simulink model "Noa_Nofusion"  (R2020b)
settings: Solver=FixedStepDiscrete  StartTime=0.0  StopTime=Inf  FixedStep=0.01  RelTol=1e-3
PostLoadFcn:
  | if any(exist('dsrtsu_mdlpostloadfcn', 'file') ~= 0), dsrtsu_mdlpostloadfcn('Execute', bdroot); end
InitFcn:
  | , if any(exist('rtifpga_mdlclblib', 'file') ~= 0), rtifpga_mdlclblib('Init', bdroot); end,
  | , if any(exist('dsmpb_private', 'file') ~= 0), dsmpb_private('dsmpb_mdlclblib', 'Init', bdroot); end,
undefined symbols (not defined in the file or in its folder): ACC_TimeGap_DecSetSwt, ACC_TimeGap_IncSetSwt, AccelPedalPosn, AccelPedalPosnVldty, AccelPedlPosnDiagc, AccPedalOverride, ACU_ShiftInProgress, ADAS_Posn_CurLane, AESSwtReq, ALC_SwtReq, BrkPedalSts, CC_ACC_CANCEL_OFFSwt, CC_ACC_CRUISE_OFFSwt, CC_ACC_DecSetSpd_SetSwt, CC_ACC_IncSetSpd_ResuSwt, CC_ACCSwtErr, CharSpd_ms, CSA_NODE, CURRENT_GEAR, CurrentGearValid, DiscIntNeverNeededParam, DrvDoorSts, DrvSBR, DrvTrqReqOvld, ECMACCInterface, ECMRespACC, ELKSwtReq, EngLimpHomeSts, EngSpd, EngState, EngState_PHEV, EngTrqMaxActSpd, EngTrqMinAct, EPS_DrvInpTrqVal_HighReslolution, EPS_FailSts, EPS_LKATorqOvrlDlvd, EPS_LKATorqOvrlDlvdVld, EPS_LKATrqOvlDlvdSts, EPS_SteerMod, EPS_TrqSnsrSts, EQ4_APPINFO, EQ4_LA_ELEM, EQ4_LA_HDR, EQ4_LAP_ELEM, EQ4_LAP_HDR, EQ4_LH_ELEM, EQ4_LH_HDR, EQ4_LRE_ELEM, EQ4_LRE_HDR, ESS_PedSwtReq, ESS_VehSwtReq, FFogLmpSts_F_Pbox, FLWheelDriveDirection, FLWheelSpd, FrntWiprSwtSts, FrntWshrSwtSts, FRWheelDriveDirection, FRWheelSpd, HazardLmpSwtSts, HCU_AccelPedalPosn_Diag ... (+151)
libraries: simulink x144, dsmpblib x33, canfdmsglib x10
(part 1 of 20)
PreSaveFcn:
  | , if any(exist('dsmpb_private', 'file') ~= 0), dsmpb_private('dsmpb_mdlclblib', 'PreSave', bdroot); end,
CloseFcn:
  | , if any(exist('dsmpb_private', 'file') ~= 0), dsmpb_private('dsmpb_mdlclblib', 'Close', bdroot); end,
settings Model: DataDictionary=HWA_DDs.sldd  RTICANMMDATA=struct('GeneralSetupData',struct('modelroot','F:\05_dspace_Work_Files\11_HWA_Project\Git_ADAS_Store\projcct\adas_project','generalsettings',struct('filesettings',struct('destfolder',struct('Name','RTICANMM_FILES','Check',1),'buildfolder',struct('Name','.','Check',1),'AbsDestfolder',struct('Name','F:\05_dspace_Work_Files\11_HWA_Project\Git_ADAS_Store\projcct\adas_project\RTICANMM_FILES'),'AbsBuildfolder',struct('Name','F:\05_dspace_Work_Files\11_HWA_Project\Git_ADAS_Store\projcct\adas_project'))),'options',struct('addpaths',1,'rmpaths',1,'addtrcexclusion',false,'cannavigator',struct('checkmonitoring',0),'show_usrtrc',0,'use_usrtrc',0),'advanced',struct('options',ones(1,100)),'MPSetup',{{}},'RTI',struct('Type','DSRT','Ver','4.4','Date','02-Nov-2020'),'modelname','Noa_Nofusion','block','Noa_Nofusion'))  DSRTSU_INTERNAL_RTIFPGA=170  DSMPB_ID_DATA={'108889',struct('BlockId','81ba8c02-39a0-4bf8-971e-fc8bc9e1d8b0','SignalIds',{{'e6dae809-112a-4cbc-98f9-354c12187ac1','31d2deb7-ef93-4695-993d-314bc5bcc843','62343d78-d15a-4a45-8693-ba2849e89479','c13156af-d15b-4771-8a29-b8e73d565fa8','cbe04a47-fa20-4770-9bbd-4a07b568eb2e','59e00f7c-c03d-4b80-a5ec-a7b536bc6272','3f246c43-0baf-4388-bea8-c24249e8d124','05e7c6b4-9822-4e1b-91fa-c2d47c80a9dc','3c91b297-0034-4136-9460-a9a71fb1b160','b0eda23f-b1b7-44f7-9430-f2199b0de4f6','d9349f60-73fd-4e07-90cc-b8a5cfade7d1','f893d12f-c8e5-49d5-ab09-89fc2cdbf4b7','b489956b-9fe5-4db2-8485-d07366cb4569','0fd99c70-4fef-4ffb-8340-8501f6b1f5e4','53dd6ff7-6c1a-46a1-9139-61ea4f9d24e0','93fe1b5e-8abc-49f2-ae51-04c114465812','9444d888-9a75-4226-ace5-9b052183c8c8','ce7a08f7-cc95-444b-9a6f-cd5054dc142c','683a3bb5-05b9-4d71-b570-d34d769ae407','6e290ea9-9348-4509-bbba-48e715a1ad64','385761be-a1f9-4d98-b926-1efaecbe94cf','77479779-8c39-4f5c-be4f-4246b8ca51ff','094c4e00-d8db-4561-82fa-1990a2a46c70','8fedcf21-59e1-4a11-b24b-5edc3eea11e5','de2ede37-26b1-45c0-988c-7281b852313f','ed4cfff0-74cb-4a5b-9058-099c9444dc97','d8a92eb8-77b2-47c6-a14b-19e5a6c1880a','bb80831f-ec06-46fe-9a60-525cce3db11c','089a9e8f-4e14-4d97-a75c-e18256b8f73e','116e4020-4c03-4eaa-a133-5105e1ad6c2c','5d390f2c-fbfa-4acc-8e45-8a78ede6d630','e0ea540d-a3ce-47e8-9630-4c2a7c2611e9','1338e80f-eb11-478f-b148-febac8b5f561','40cb9f5e-abe1-4c5a-91b1-6a21a87629f0','f68eb2ae-9d65-4ce4-8ae6-7911307f53aa','90ccc115-d294-448b-be51-2f0d4ed4df75','d061fb9a-9168-48d0-bfc4-e7fc980285e5','66fbeac1-5405-448b-aaf2-b3b4c802c6b3','18d32c7d-1106-4865-b268-b9839028e3ed','68ea3199-eee5-4804-a61b-b9492c15cc17','251bf7c6-0b5c-4442-bed5-124eaca4f0a3','5c44ff7b-7cde-47e3-997c-d7e4d571a688','a318a3ac-fb11-4e42-abce-b283a20da434','8ac8bf9e-cc00-4453-b1d3-1d8cb9e4d5f3','e889ec5a-b6bf-4115-bfb4-789ddcbb1b39','843277e1-c8e1-4956-bb5f-69810b3fca13','8015402b-cae2-47f5-b799-3258863f20da','967f47db-98cb-4b9d-8737-8d02120e8039','408e6371-4b24-4e9e-8575-3f5fd9116599','0add38a7-641b-41d0-9036-40ff81d44c7c','42c9e777-d5c1-4821-b220-ee42a71da039','1eccc895-bd9f-4c89-9169-915b3accee5d','c32a22ec-25cc-4381-9457-3401f3ef52f2','dadafd58-4047-4fbe-8c61-d0d4f2e948e4','33df5bd2-20b0-4ead-bd24-c6cd609c4787','a6ef951d-803f-431b-afeb-b8db87ab93f4','3d89e518-12b9-4d0d-90f2-936f61a4e4f2','f4fba2eb-28a8-4b3f-a3d3-e6a85bead6df','1bbb28d7-2fef-43d6-b55d-c5356e90e304','46c1d4d9-bf71-419d-bdfe-9c3255f570d2'}}),'112056',struct('BlockId','6913c789-035b-4c0b-bbc8-df30b7210019','SignalIds',{{'6e67b619-d0e1-4489-8e12-cbb641b6930f'}}),'112939',struct('BlockId','bd32a928-034f-4d93-abe8-55cc1037974b','SignalIds',{{'ed378323-8937-4e58-90a7-af861033d965'}}),'112945',struct('BlockId','c5ed9ac9-a557-4e9e-b1b2-178e2ab00d3a','SignalIds',{{'9bf7ab65-611a-4ce6-8553-94d5ebac5e02','125861c6-7b90-4e8d-a590-5d6d82b8a9a7','4aee84b7-a55c-4fa5-a4b0-5c93a3e16834','bd31e0e7-f9ed-4a3b-9100-c48940e83979','f56bb652-89fc-4dda-9d9a-1212207cf3a7','0e2341be-0c6f-46b5-93e3-ba9acd4843ed','91d7f4b2-8cda-4163-9f74-f5dfcbc91f25','b0e338de-3225-4d50-a22b-4e417233ad31'}}),'113655',struct('BlockId','cf6f5b87-7341-43e1-a3e2-6f8acef19396','SignalIds',{{'fb5a5d6d-2525-41ca-b3f6-99d6346c30ea','ae8d4c22-9733-4a6c-b1e0-ca44fb9aed0b','e1e4207b-e7d4-4434-90ef-6db7c466bdcc','10f1d399-af2e-4f78-9956-e1f0397ac4ad','4b9c207b-4222-4e4c-a939-fa1aa9ebbaa6','60cb540e-4d8e-4be8-b719-3a1a079b86f3','7a6de52f-e056-439d-aa5f-cbeab7f01795','aef0510b-cc97-44dd-85d0-c0d01358d9a8','81128469-f06a-4068-854b-26757f57e96b','bef5065e-4128-4abb-aea9-c2d2196590d7','71c1176d-d27b-4ef0-b058-205366da91eb','a3f3e7d6-0f7e-4984-a2f1-0321a3d087c0','b8f4f6e5-954b-4f58-98d6-66ac20499b5e','1b7b5941-9f2a-477b-be19-44adcd6fa043','0aca1d39-c4d5-45fe-b4c4-9737676b57c1','e506b680-642d-4f46-a400-b635b37ea192','c25a201b-c2c5-487a-9976-20a56153ab24','f54c3c26-ca72-4882-a2bb-5b3ec148117f','92e7bc4b-0bc3-4bce-8cc2-cf8f985c98ee','153941b6-b33b-4fe1-a541-d5210f1cf000','89f9b2c0-1175-4586-8022-f8668d534196','2e6f805d-9e7b-45c9-86c4-bb39c1b2e16f','812564df-09e9-4888-95e9-ea67c66976c9','ad32a513-90be-4e6f-8d45-3c98afd525bb','6bf7cf6c-3db5-431a-aa46-6683249e747d','d0d3bceb-ccfe-496f-bad6-d5b74e8fe321','28d4a00c-23a7-4c5a-a473-39ff0814a4a6','cb76da0e-2e0f-46bd-b5e5-f0a979fc9b56','dbfa4afa-9e88-4515-b868-620e1ca4efcb','9069fd4c-b476-4ee9-ab6f-15984b4dcbc6','7aa0c299-49d1-4bff-bafb-8f8a0898bcb9','41a89758-675e-48c8-b1f5-09ddc1e1d587','88f85f3d-145f-48e8-bc36-fa5a99545391','17419447-9e4a-42e5-a167-9f836768a643','7afdf13a-9d25-4c4d-8007-226f9de8ca9e','59952105-0e5e-4efa-ab7b-4572f1fda11f','c96169fe-d7f6-4165-b1ad-2f304687a6e6','24738832-79b4-4001-8229-260d8feb4113','86b2b6a5-44b0-46be-a990-c83a6a69628a','440d9c51-e2b3-4545-96e6-96bbb804c01f','2c6095e2-8169-4ae4-a16f-79f403295a42','cadb492c-0473-4401-be06-10367d0aa2ef','4e68f589-c74a-49e1-ac92-78db45f8ef8c','77831aa9-1b69-45e9-bbee-3b14b9e34578','f5305063-53ac-4dc8-9054-75ad211f45d6','5ac2eb62-480b-424b-b3fc-c0796833d037','baf4b3ea-4bfa-41be-a1b1-216d8e77a452','5a3c4cf6-1180-4e87-8a7b-237d3d652526','d1686968-86ee-456f-911e-0d6de43751eb','166edc4a-1ea0-4644-9293-bfcbe463d6ad','20e7c49e-9ca2-46af-acd9-1232cce0faa2','2fe2470b-9364-4832-b69f-2e5d9d6c017d','2429babe-f40e-4f87-8c9e-2b0729d1c86f','36be9472-502d-461e-af19-fcd14b7c07d0','4c6963a3-b37c-41a1-b24e-c4c74fe8b70e','017cf1c2-cd81-4f79-8072-322d3a102b1a','00c4aaec-f88f-44fe-9513-f362b17663da','92dd9569-6fd6-4cf3-881a-10befd4b7a04','110c0564-d01b-42f2-8faf-9704e9fd9cd7','1a8a2e8a-c290-465a-a25a-8437cce6393a','98a367f9-c024-42c5-8458-b1267635b2fe','9c1fd1a9-d357-436b-b199-147a0771b5d9','70dc3328-065a-48ed-abfc-2992969b08cb','0fb59dfc-84c6-493b-a389-3fb28a6d9fe1','0f4a0327-4eba-4d80-9017-dba17db1341e','8cc82210-4aa3-44d9-869c-a0209d9ebe66','dc67f717-48c7-4ce0-9dcf-e91aac01697b','01d17e0b-0a8d-4114-bd9c-6b82437e2631','c90d70b0-ad54-4755-b5d8-75e9be712e4e','cf4155ec-ad34-476e-ac0d-8e69f7d22b3e','b127da2b-81a2-492a-9a1d-7dde354402b7','7f843f67-d354-4c08-b6af-2ff3e43672c5','f4418185-a712-42cf-8d77-411d214ab81d','59e3a284-6d51-47b6-969e-f6b4d8174f3d','b8e8aa68-fd96-4202-895b-fd402c9a1341','5fa25c56-4452-41bc-acca-9957ac1b4103','13cf6133-db9d-489e-8b0d-61e9b3419fae','71c8cfac-5807-43ef-a652-22095fc79882','15c70bed-afca-4d00-ae5e-dd51784e9f61','aee1c38c-6fb3-4ddb-a252-226dfbfb6422','7168a0ae-fcdc-4521-b98d-6a441943bf9b','5dd8b7ac-f364-465a-a93c-c9343301ac44','df0fde16-8f04-458b-a7c8-834de1c017b8','3a947018-17ad-4272-ae69-eecc79aa5a06','cd4f05ea-2a10-442f-b08c-e22eaeb8013d','cfd99e2b-6a05-4d37-bc51-f59eebfa85f5','aa629df3-c01f-49de-b905-c90313b21dc2','22d01045-bbb1-4d02-b693-732a6fc069ae','c48275b5-fc3c-4e5d-a241-e78a85a3ad8c','c56eb02a-4f36-41d4-b430-a4b28301ef5d','bae3b75d-9e5b-4327-b68f-a846466c9a9f','400fe431-6ea0-4473-a63f-9ef8d119722a','02db0c0b-dc19-45c7-8838-2e3a10b74905','48aa7831-7c07-4a00-8123-89d3d6d7594a','bf73eca7-8306-4a9e-b009-9c4be8fbd534','d538498e-adef-4247-9bcc-456a97e2113b','d0492371-75a9-4227-9ab1-7e8aa07d4fa7','115c5825-4fd6-4e7c-bdc5-7fe3051c0051','ed0f82ce-ae1d-401f-a42a-e322d0793cbf','aa1610ed-12f6-4ed1-aae0-3315b1eb3f84','63583f44-8eb9-41d6-b0a7-68eac98b41b5','c96f8dbb-26c7-435d-9572-792809250d8d','f1980f8c-e4af-4d1b-8b98-9d32743e8941','a4369ee8-1173-4fa4-9ee3-615cb3251022','90c0388b-7c95-4d96-b447-7c88a50c7164','173dbe10-46e5-4294-a3ec-3e0e30e5a6b6','529d5fb7-0bae-43e1-b06c-704af90a34cb','3c503139-d85c-4ae5-a8e2-dee622a6f9fc','d16ad6ae-6cac-4f83-aed0-121895af10f1','f6e64590-8c21-4a07-bb10-99a1519377b0','ac732596-2512-40c1-b579-190acdd8e089','9816bf99-2d8e-44e7-85d1-d4b65f13525d','fbf136a3-9574-45df-80c7-da1f97b5e35e','a12166d6-84f5-4f22-8379-ecc27ba6ae9c','55221980-234a-42fd-aec1-f26d2630223d','f2f07aaa-464d-4e08-bbee-41e72004ebfb','03cc4663-40e3-4a19-a510-51aa2d1d5c81','c6d48439-bfbd-48e6-ad19-a014aaf6d7a4','26888429-99ef-40be-9301-8bbe11f917c8','965f7110-f95b-498e-815e-73cc2d6d6525','f2d198cc-4bd4-47b3-8c41-c7e19266237c','0eb6f2be-800e-485c-a213-fc91674a796e','14566c8d-2b3b-475d-9ec4-34982939edda','b1531aa6-8f0c-4ac4-9759-53039e63bf9b','f03e1eca-afbf-4e5a-a201-deca4b0487b3','1fd091fe-0624-4b60-9f3a-d13954dedfee','f86c37b6-0788-4db1-b32a-02556a39e0dc','eb622d94-f642-41f2-ae16-5748dc9eca3c','f552e8bf-3199-4d81-be32-9694985eedf8','89df7002-4106-4bc4-8041-9f53e3d16869','212e5966-27e2-4926-a8e7-97e15aa44966','d800a550-6f5f-4611-be9b-77cb4f1d501d','7c97f8e2-f557-439c-b46e-1b618bee852c','ba8c36d0-0984-4461-a832-bfa5f921dfb5','06934513-6eda-43e5-9ba7-043c69abb13f','00daf677-ba6e-4866-aeb4-cdb14cc8e0b9','078b0d6c-c412-49d2-950e-bbe655339b57','239e3cc7-790d-4097-9a56-e63ab309039e','66b7e7ad-a98f-4fbc-9e25-0dac0827d61c','315dca2a-b23e-4eb3-9e0b-52140b0168ea','b6365e66-fb75-4629-937b-80d218075377','9b529c23-3902-492a-874b-28d45a35fcaf','9353632c-29da-42c0-b854-eedca60acfed','b766848c-b98e-4e0d-8440-f607563ba8f6','794edea3-10a5-4aec-a36f-e1459d729f91','43984543-8420-4c46-a3e8-2d784edb7c6b','ab504fde-7461-4895-9a45-667a2b575a53','6bc6eec9-68dd-49c5-8569-ec45206b9a33','bc6a11cb-2543-455a-8027-a475be328250','8cbc4c4c-4bcd-4e64-a3f2-8b1ead7218ef','5007b9e2-cba9-4a18-8f0c-5063bf4128a5','2aad26d1-b92c-4482-b26b-b7acf4fc1308','95f5773a-c7bb-44a0-a919-27ddf233286b','9e8d56c1-5230-4c79-9a8a-dc1b7934edc1','60a91cf0-0afd-46ad-ae58-fb1a2eb831b9','4c89a1ec-5f31-4d14-a287-1ccabed8a64f','c7b205df-5cce-4a4e-ba20-1c4bdae77031','c5981b5b-3b20-4a4d-9505-1eac419a8f7e','6f213db0-4ffb-4883-a14a-5b45ff58725c','2a8d3af2-5809-4f7d-89e2-80bde3f8ad32','ed1c9b94-0fa4-4bb0-a2fe-4bb286367636','4a796490-b3d9-4bba-a58b-74691b8b9c45','3e10f08b-c794-4285-b936-32a0f1309fd3','83fda9a6-ac79-4c7f-9344-c587036b236b','1cc4289d-4d7a-4fe6-bdb5-f78a307c0c9f','b5275e4f-1cc7-4a3d-b6fe-0b4189fb04a4','2e56446c-c333-4276-95a7-367f5c85c84f','e3b40b68-b9f0-4ec0-9836-b744d2e81a25','6dc5b3ee-34ab-4f3b-8a90-542aca188307','19fe3b5f-6175-40e8-91df-5be10690c48a','bcc012ad-6a8f-4b49-9a64-37954720d3ac','140a9a36-67c9-4b06-8b1a-2c2bdb5987e8','a03085eb-5191-4509-9a9c-9f34d876ca3b','5f4143a3-b004-4871-8e65-77221395668b','86ea935d-0a1e-423b-bc47-02ae6b6a212c','6baf03a1-b91d-40eb-bce4-0ea061e1b9eb','54d848f2-396f-4317-bd62-e251125d29aa','19f4b235-e4a4-4b72-b459-b188be453e53','5343c8e3-0bf6-4584-9728-1ffdf78a1c68','60ad3be9-877a-4b12-844f-f4d858a22658','adcf0bd6-8038-4d49-afc5-721d0c718c63','fe594a46-7e27-445e-829e-e368b2766e07','34b661d0-722a-48f9-9697-2658f24a22b0','06588917-d49b-4cf1-8374-3b911c00cde5','5c34855b-78d4-4797-82d5-4cf4fb5597c2','08cc61cd-138e-4046-a793-e08ba6951309','a0299fef-0823-42f0-8309-d7777acbc38a','e0a15817-9b40-4e70-969e-86236bb9f230','9c56c4dc-6508-438a-b106-2303bc6695c3','dba36f32-39ac-41b6-9312-d45812cf79de','2d770f77-49bd-4944-b036-dceda0114cb0','d649385e-2647-4aa9-9434-450787e207f3','aea55e49-0b3c-4de1-bd15-8d3a264bed41','bce569b1-2dcf-474d-b5f0-eaaba8306cd3','188b79e3-5a90-4177-a30c-289bee269920','bedbb28f-052e-4eaa-a863-033c9bf7d025','5061b3f3-9e4c-411f-a66c-77787e28b206','16d831e7-1cc8-4971-b147-7b6dd9f1e240','602d497b-3413-4be2-a3ae-0627235695d9','b5052d5b-ffb5-4989-a31d-1768a8ce989f','a859376c-290e-4574-ac12-3aa5aeaca50e','64528274-e7f3-4fe7-823e-a549b5173330','e7e53007-1b26-4631-b4f0-90657a77a9ca','5bf9ee21-94d6-40cd-a889-88d08a7a87e5','9a38031f-a864-42ea-8e2f-b35739f9c0da','e7cb1bc1-e249-4a65-b9af-f693524c4367','b5764df3-fce9-4fba-babb-0c3ebb3c0ff9','67fa94ff-08fd-4a02-8dfe-1b7ce6c0e586','1d55abc3-0a99-4ac4-9732-7251d21b101b','03ca9ed0-8b4f-4eec-9e40-39a068e3fea1','692ec90c-8e9b-4031-84bf-366e08f2da13','be841484-f40e-46bc-9894-07f688db3a45','47930925-babf-4f1f-abbd-2ff62ce38353','64ba39f6-08d5-4ebc-9f32-4871ca2ba973','f69b6ed1-4854-4198-b013-d82baaa470cb','23d63867-9c16-4ada-a94a-83a465157190','b20f84ea-82e2-4769-80ec-cf58304b0510','8ecc5c53-55c9-498b-b349-bf6ab70d66eb','e6a2b593-080c-4bcf-8d98-d1bebd736166','aca64f4d-8f9c-4329-bd12-0bf755dcf6b2','541ff6fc-3cb8-431a-ab40-7a0072923e88','6a467d04-2bf3-4197-80f5-111fd640a6b8','388c2691-3673-42af-a5bc-3881b21e8e4a','58794cec-c59f-448f-a084-9559b6fdbc3c','53969dc3-67ba-4150-8c28-2139dcd36ec4','b047deac-9e80-4433-acac-cbf23acc33d7','893ee9b8-2597-4f15-875e-3c3b30945b0e','e6ddfd0c-2f8c-4b29-8e36-05c9546fe401','d98547d0-f670-4ea4-b98a-9385d86c2203','3b07b467-bd0e-4454-bb9a-90d280d34652','bf33618c-d18a-466d-a60d-60ac0c9409f1','775e1b57-a066-47f3-8cff-496f01feada8','eaf30c55-fe96-4594-8469-a63fc7e3cc74','c79fb195-18a4-44a3-ad68-cec237ffcfbb','ed0574a8-f84b-402a-8e0a-efcd9c69260f','3be3ed0e-9f1b-411a-a012-2e23b6931244','9d2f5e3a-9477-454b-bc3a-5f933716ee7e','8eb59546-6e82-4fa8-bbb0-53768d49ea0f','e6d25c3d-5af7-4b2e-a6ea-e57a6a9082fc','ccd97ab0-e4ee-4603-94a4-f590f332a0a0','36ec9cb7-c0de-4262-bfdc-48de79f1ee61','efb2231a-227c-4972-8174-d25c5af76b54','b8657e90-21cb-4618-9e22-eaf8199bac0a','ab860674-1233-4d97-baed-976b22bdb396','86e17527-957b-4763-8fcf-1efdfe4bf5e3','8976db8a-c2a3-4c2d-94d2-ed11fa88995e','fe62eeb1-fc5f-480b-8fcd-625981641e99','98479ede-546b-4ce3-9131-f97f4f44b420','455c1b0e-8996-46e3-8765-b54392466814','eecd774d-9fd7-4e12-a69f-9158539ea43f','64e999d6-79ea-4c70-9691-0f70a2e71a3c','4f106621-85e0-43b0-9a07-97ba4e62a39a','ded46c33-c816-40c2-a14b-acab78f6194b','71b6d7f2-5494-4e5c-b708-3acce932e9b4','85390b41-ae3e-4f17-880a-2f84f64fbdc2','80ebf2f2-1e3e-43b1-8573-c57fb60b5bd3','fcb015a3-dcd9-4ab1-ada0-d5f9b36f4f65','f248bf76-1aad-4be0-8fd4-444403bf160b','c9bc3de2-4dfc-48d8-9321-9541506ead43','04f847d3-9b90-44fc-8000-a37f05680c68','e7b03f62-ce12-45f9-be9d-dfb471f40d5a','c756a44d-6650-48dc-9fe6-4644269bba21','52c0df97-4f48-466f-b21f-e5da70460700','8cc9b746-8314-4707-8eef-133a09ac600f','10ac6bb0-54ef-4036-8bf1-e4fe44cb51cf','f01401ff-5618-4763-b3d3-05e925429136','099b9e22-bfd9-408c-8a69-da181b5928a9','8beb0841-bfeb-4414-84c9-5837efbec2de','7cd0aa18-ad0e-4f83-b529-0b8b1edbda58','5a1ac686-8048-453e-a8ce-8411f46fbd2b','f6b089e8-1714-4554-8c6c-ae277557d6b0','7db72d27-357f-4165-a42f-ca134561865a','46b2ee33-2a46-4639-aa6b-31804f0eb79f','bea151a9-9470-4a1b-b4a4-d6ee65cf1a6d','9d8e8e72-b826-45bd-827b-4da7309ec902','524ada8e-5caa-4eee-8660-8ba270afed3d','1fa5b50d-1d22-4e8b-8caa-6099f0365943','39a397c6-6b9e-451b-acd8-22592c114d6b','831036fb-a144-4ea1-a442-c82e3144a6dc','7c0b476f-8e10-493a-a767-b34803d3f906','6d8c8cf0-32d3-4208-99f4-521a6d0dfd21','85e195e8-f95d-4695-94a3-91a9453eda3b','d8375b92-e629-469d-80ee-3ffdb94748df','0bbd0d2c-c3e1-4dde-be1e-7ddf6f726146','1c0b1a90-2d20-4696-8efd-9f1a664ceeb8','5f40da94-a4eb-474a-807a-3dd0bcb36476','b76fda9b-9022-4987-b854-ac9b79e9de0f','4d85e715-c5fa-462e-a30b-78a2070e182b','ef6de948-8284-46a2-9857-334cf6955462','2c5d1523-c178-4d85-b549-a99b3eb458fe','7acbb973-8a66-48f3-95c7-0dfa2c4f7a67','76e94742-1173-4778-b958-9a8af732c510','39639f0d-b40e-406e-bcb8-1115e41ea694','9a0f6033-a915-42dd-b369-6715e99a36fe','1f2532d0-eb1b-4d5d-a15b-9633a6182d9e','8ee71d14-3ed0-4cef-bd81-023e02cfdcf0','0425d3eb-89a2-47e4-b191-c06301e3a22e','7bcbf577-ef09-4b1e-9393-641a8fd1db45','e972e0d7-5969-432e-9c13-ed69ec3ca15a','8cfe49fb-b648-4e0f-997d-a4b705c3dfcc','dd620b21-6e46-4537-86c8-a85f7d964964','7cdddb47-3327-478b-b5b1-b24a0d265f98','e664debb-f201-4a07-8c66-4d8d4f01eb58','046cba93-85dd-44c2-9d95-fa8460327d8e','4a759089-51fb-48c7-9769-fd507bfa1c31','f30daca8-16cc-4116-b5cc-4c4d0b2485ec','a875cfca-7d4b-4419-861c-f840c8cecfc0','16bd4e98-1a2a-44a3-940e-2c3536726d54','8fe58d6a-48f5-4feb-9712-57cfc475acdf','baa4aec7-cfce-4df8-94f6-22f72c2926fc','2581aa2c-fc12-4834-8dfa-72962f7bef6c','73275ce6-7ae2-4eb9-9ad3-4a4dd83d789d','e4177cad-9e1a-4600-90af-08e140daa85e','bbcfdb84-f26a-4496-829f-5b524010ffb8','175863e6-df8d-4788-aef2-ce778f26e881','ce0d4b96-7971-4b55-8dc6-4be533990611','6d43a9d9-4fd9-45fe-a8df-2cd804531c4c','b1ba8b2d-b9c4-4d26-9419-a0dcb9edce61','12954d0a-2153-4a15-97dd-73a136ab193c','24bb01c3-307c-4919-bc31-35878986a0ef','ff983d94-9084-4828-86a2-548bd2a52142','306ccbaa-6f5f-4218-96f5-6c0edfa4c4ce','933a7bad-468e-44ac-8774-297e3fd6bcc5','2a7b0ee3-28b7-4249-9879-e4ea819ae9b9','a7794c25-04d8-458d-9659-d0900b7d76f7','2dde5942-bcc1-4378-a291-1686e740d175','b81c4a5c-cc0a-4157-a286-0570c1f57373','23d6a580-0376-45aa-b2f3-21d12703d075','c2def773-7c89-49a5-9656-f74c558a69fb','f9d6d86f-00f6-45b7-bf3d-642740cb4d34','985ecc94-b959-444e-ad73-ca286a05a0e3','1f64d2c2-eac4-4ba3-bd38-eb050c680b29','f951f26e-dd6c-41bb-8c65-411294b11f18','71a53544-65b2-4317-8643-eb8c723f475d','43afa3fa-6ef1-45b4-acfc-b905363f5a1f','2bee269b-6354-4dc0-9cab-da7990c363bf','d8008aae-9797-4911-9c7d-941aae07e1b9','ad4a91cb-3b80-4ed5-8903-2cdecc13640a','03eaf39d-7ab9-432e-9dd7-392ce605e292','469ff205-0a87-4385-b8b9-cf297be9f9d3','9d88b864-d7d2-43e9-abda-a199627a1c3a','f85e8719-b835-4ac1-ac53-4f8c0354d903','5035874d-2848-42a9-8267-e42c6ffebe9b','dd323b45-8533-4388-978f-13dcfc1ca4dd','e1ab5525-eabf-468e-a93b-891c5e3b3232','7aad39dd-f2f4-41f8-af53-33b4b67b233b','dfacc862-6abe-4523-8a7b-5e45039e9a02','cd2ba88c-485c-4d26-b32e-d352de9581d8','4a87daee-f3ae-4344-abbe-a3ac11380b5d','6c863c5f-ac8a-424b-b2b9-3cad00bc3dc2','6ab98864-884e-49f8-9ce4-390f4f328012','3e33b112-c9c2-4a13-a5df-d3f630b39a96','f535ee26-dd67-4a93-a192-fa1bdced81d1','c6672b46-032c-4c7b-88c8-ee022f747061','9e5e194d-cc6b-45ca-b097-2918f4c7c1a4','14ed2d72-f7ca-429f-94e8-eaf8fb4b9ada','62f116cb-c0e6-4fa9-a341-ca2d22d4e417','0d8ed1d0-cab1-4595-b27e-36cb0d2318ef','07734f33-025d-47b7-b0cf-8cf3db659c1f','d497876f-5146-44ef-a456-b0f1f106e54a','d4774d69-ff58-4107-9c48-01f0346f3863','58094a15-108d-49b2-b3b2-7db860c594ad','97077705-a187-42e0-a62a-49d9ef388a97','1a386dfa-1cdf-49ca-864e-ed1d354aa34b','ecaaf82b-880a-4a91-af87-61a72c059eed','03aee385-64c1-4271-8386-df72e39779ca','1b629ab9-72ad-4595-b45f-ea8ee96006c5','8d98af7a-c034-4da1-9390-dc5bd0b57132','1b491f59-26a4-4979-a568-b4dd22586424','c1b715e3-d427-4ce5-821b-9fd5198f426b','6370c40d-57df-482b-90e3-d307c6c8eeef','eee89dd1-5b65-4aef-ab52-a5f8fa1ac4b1','bed978c2-1ac0-4ebb-8765-84d082bbafd4','97ad906f-9c9f-443b-9fca-49c74aa248b5','73ce7988-7d70-4411-acb6-da032dee2a0a','e7667fdf-9dba-439c-9dc5-2207472cac42','3ed46ec0-bd51-4e73-911e-6653eb6d3f57','6d8f67f6-b707-4afe-a8db-c0922108ce50','fedc2364-b159-4118-a69c-608448574a6f','3f6b3971-1edb-4b7e-bf65-4b7708d97251','9aa7c382-a12d-438f-8a09-858e2d819d97','35e43c30-ebb0-4e8d-84fd-1df3498170d4','bcb5f7a3-6417-4a3f-9f08-502db4c96922','3d12e05d-3a35-4a5c-b1f3-ce750a37a37f','61f58b0f-bd5b-4a6c-bfb7-21da4434ca2e','004b1744-3784-49d1-afdb-d1bbbd89db23','fd365cae-3646-40e5-8b64-49b0a514e744','f12b7859-93ad-47d7-b778-08b35515af1e','c1290511-557e-4648-b4f8-cad2e85be107','9cedc079-bef2-4bf1-89df-c2dcf5b3c280','82bd5b77-f41a-4265-a96c-2f6cd538d380','9db0f220-f33b-4415-9664-45032d4cbc2c','e7098033-df4f-407a-9ac2-97d5af91084a','b849b30b-a487-473c-aa9a-426282fbbcf2','0ba9e83e-1b76-41d6-8e64-6ed1d1be4668','bd8c6b90-c04a-4a2b-b726-a49dfeef42f7','757e2df4-19db-4522-ba8f-dc03ce29dcae','ab9dc673-331e-42ea-8b14-86e44d9b8e35','7c90f166-1d4a-4655-8197-3d8dbe935965','a648cb07-2aab-49d8-8679-a384bd0d3a53','c2a7885b-b256-4ddf-9959-d32f63b0936b','ef68b66f-aa01-4557-a706-f3fdac7ab903','7ce622c6-0965-4c01-9bcc-6f0bd5e77c3c','ec59f638-7a3e-47b4-ae3b-a2ace313f6a5','b65978b6-fd0e-44cf-a75d-c43d297c982c','77ce9763-3765-4d4e-afd7-22b36e684e79','ee2b9016-5cb4-4078-8d6a-147b7435587a','a1301744-4508-4733-aab5-72aa11aaa2b5','5926a83b-0259-41fe-a971-de014e905815','51ac0682-5edd-41ff-91af-30a44f078d70','070ff71f-113f-492c-b510-f6cf1b65fc77','c1d9762a-5e41-475a-991d-26de0ac35969','ef65316c-36ba-41af-83f0-4ef9351f32ed','09e6ece3-dc3b-42a6-b1bf-512e15d74582','3f1c0340-dcf9-49e3-b7d1-3476f2943ab8','0ac26106-35be-41a7-b1fd-7ce7a0d8245d','0b658e1a-21b9-4272-aac3-3722bdfb297d','e565bc53-3fe1-4a44-adf9-ebec7f459566','b6dfe945-a283-47ef-961b-81b1eebf647b','11951749-523c-4ae7-8ecb-92bad7cb8061','eecd629f-9f20-4f86-a4d5-14c6a934a78e','819c048d-92a1-4c31-862c-940e8d3be9ee','35bcb929-fd6f-43a9-b541-281ae7948175','8734706e-5c3a-40a6-9805-fc57ae5d7936','44b31e51-9bdf-4a60-98ae-283937b0b951','af113ee7-f36f-440f-a9e6-c09a524de4da','880b51be-8dc9-4eb6-aef7-f5858f9a0101','fc729efe-1f08-4ada-b36b-cc9043232b4d','f7129efe-e766-4363-81e6-c8d494debcdd','92f10edc-462a-41c2-b558-54e178699d01','b4a4aebc-e2d3-4c89-89ad-c33211611583','2f469cdc-da00-44da-ab21-e52afd88454a','2a777674-b740-43c5-b2bd-0098c234417a','b6c767eb-501b-4f8a-bfa2-3853c8a8bf2b','12504ed2-84a8-4a18-b1d2-3b7a798da722','d7de8f4f-3939-4c2a-9cc9-b385407e6445','cc1fd519-9e95-45e9-92eb-a9682942f77a','5c3762dc-464f-4878-9f8d-09e052620d4d','20191a9d-3f53-48b2-a029-ff3cfc487637','e56bef79-1d4b-4ec8-a5b0-0137475c4cce','4177b81d-b877-4551-9519-dd78cad2bd98','0f6c7aff-26fa-4aa3-a752-59084f8e5854','574d7bc3-e642-40f1-9195-711319ed2921','e188519d-a655-418e-b59c-52c5bedc9f4c','6d81b244-27c5-4ada-b6d8-fd407b6cf666','e18f0370-93d4-405e-8488-6ab967af7366','56591c66-ba21-4450-bb45-ab6c1596aba8','4eee9bab-c004-48a7-9272-65360ed8830f','2d89c8c6-c706-409c-bb4f-b924ac39ab6b','5273e952-9022-4675-9270-067109e898e1','c4084d0f-03f4-4c21-9eb7-25b30f4541a8','027f0eac-088a-4b8c-a74f-de626fd2fa06','32da9c63-2094-4f58-8c78-0e3721b8172b','1544d765-c339-4373-9c35-29d89606f15d','9cb587b3-0a7b-4ef4-bb32-bf47fe397c60','dc356749-f481-4e6e-9202-1f5d7b39f06b','ecdb50d0-12f7-4543-8ec9-83ca14be80e8','b6eb5342-0336-40d3-bd1f-5426bf8fe6f9','92cf1d7e-5afb-48c9-9635-691c1b65c8f2','f42fc00a-ad8b-4665-a4a9-e2a9939018e9','987dfc89-d9fe-4e17-b19f-17fcbb78978b','46e9915b-1914-4472-8ea3-6c17101839fb','239d5e07-5f1a-4383-8ef4-cf25ba6dc94c','c7e7cdd5-1bb5-40ba-b113-b56d396543d8','823e6229-f789-4b8d-8bd0-5b8ee5520214','b75e855a-5838-4a12-8a5e-b32c13cc419b','943fac50-50d1-4f7b-8c70-51084f8ef9dd','b37bb84b-0cd5-47ac-beec-d8b522d29dac','576077b6-c671-49e0-bfe9-824ec7481716','64103931-2a71-43fd-b9f2-48a0b5871437','f7091461-eba4-4f9e-bb42-11eb2d95df88','45150054-ced7-4afa-b3a4-2cd781a8b9ce','2f61fada-842d-4e4e-af79-a6ac2a2ba400','65c37f65-c18c-4567-9058-7eba2abfa2cc','c5a74d3c-c00c-4ea7-87b8-a14f91041339','9e5dc19a-65cc-4e2c-95c7-1d0b04ad19f9','91de52f7-dca2-442b-ad26-2dd522638f12','7d9de354-d9b6-494d-beeb-14be90ced829','d83bed1b-af46-4b39-9ed2-0f9e1d9a0ec2','b1184f42-e4ab-42f3-8a9d-df22f7c0ce8b','c8197ae4-9605-478f-b2a0-6c27756947b2','b10c85f6-099b-45e8-b447-48ea0b446790','b1c62881-b8cb-49e5-bb97-8149fcbcedda','f8f0b030-500a-42ad-9e81-9e12b49067ce','8ce2fb07-d75d-4779-96cd-d6077e93d431','d612d624-ca54-416d-973a-68e46430a5bd','69411ad6-4658-40a8-bb22-02642bf01d42','e64b4e57-72f4-4f1e-b3d3-e63c2409c1d2','da45bd3c-0a01-4145-93d8-d155dad9a4ca','88c38dfc-3ed2-4ec9-83b3-4491e0f52851','44c709b4-ecfb-4fdf-9b6a-c2d603d5e3f9','788f41d2-121f-4b7a-95e9-da80b2155230','4b78d830-e41f-4d67-84ff-28d784a67aa2','3515df17-5415-43d0-bdef-157fe533bb75','da279f01-dcbf-43e5-9b18-7cc6437c9749','e273512a-a3e1-4fc2-b6d9-b81189ca86a4','cdd9b274-01e5-4f50-85f9-856c9a2b982d','b180d54d-710e-40fe-8790-de5525cf96e9','68b3de74-32f5-4750-908d-fa35ea1f1c78','6322126c-4c72-4008-9e3f-4ee601a439cd','5b2f4177-42d9-40d8-a9f9-7dbe59dcae12','c8afd3f6-674c-4e25-b970-ae508c5fb65e','e24a30bd-aef8-4275-86a9-e6e75f4b2568','2b175393-7e5a-434d-8a36-896830925fde','fd29e8c0-fd72-4b4f-a58e-654ca6b51bcc','8f1edbc5-2c0c-41a0-928d-04eeb971ed72','4551c7aa-5a96-4dde-b08e-baa4be61c895','8c3a43bc-a70d-40d7-8f5e-281515319d4c','62b8b1de-7f1a-43d6-8e7f-92a2db39e971','4de0eb82-ab31-4cfa-b821-85276cadb198','3968a5c3-1baa-4b17-83b9-59dba80baff9','b7e8b01b-6d01-4a6d-8b89-f4b46543ba4e','dffc01b4-1b71-4aed-91a7-4704503cfc73','a0c3ed83-438c-431f-a324-8ab243048674','5532acab-b1a2-470d-aa15-d763e9f121f9','c10990cb-591e-4a6a-b8c8-a39d3c1afe45','dfd968cc-490f-44d0-ac8a-3eb7e8663a23','de68f977-487d-4fa5-98ee-d9cc5878bf6a','de66ccd8-1865-4823-840a-a2573884d492','be92ce1c-0112-44f2-a34a-8902b17f637a','eb665b99-9eca-466d-b538-ed1d1fdce1e7','1f44b71f-3f68-4123-b591-456f67efbcfe','9b067471-071b-48a5-a7b0-a42809f0f257','c25c6a82-6c32-46f4-9b5d-e2feeb049b79','f79cdb63-234c-4282-9061-aee8f7e55cb2','41172e2f-670f-4287-8dd3-2f28bb16c2da','013c5643-02eb-48a7-9975-846d71ceb630','e7bac6b9-8814-478c-a7b4-34b0daa02999','1be259bd-7e50-40a5-80a5-00f4f4738eae','3d400796-e57f-4059-85c3-a21b7dd35df0','11d9d554-5a6f-42fb-ad4f-16a4cc5df26c','e3e8f344-af1c-4403-9d58-55d61a924f05','c167a746-311f-47ed-aaa8-85a4476c478c','06d156b4-fb2d-4963-b425-744647a97132','51763ae7-6f28-4378-acb0-7ca3d6ce61ba','05fa6e5c-539c-43f5-b02d-0ea5cf80dfae','4f3cd536-5e5f-4b37-9cbd-794e763b83c7','be0724cb-7ace-4135-9e52-8448d56bd7f5','e9b79aa0-d50c-46f0-8b3a-42c903b85604','04cace06-a62a-48e6-9b1b-5f5396979309','9be7cecb-d113-45f6-bcbd-70889c4aaff7','e27704e8-8f23-4488-814e-6f0bebb31515','f649236e-189d-4833-b935-bca5e0fff521','3e76bab1-9107-48d9-914e-cb874dc51a44','53f8c50c-ffbe-43cd-8f43-041b179d03e1','a5a73d66-d237-4ddf-aca2-954ee4a16cfd','1531cf21-eb73-4fb6-bda9-8067a1e5e217','642436ad-5df9-479f-afc2-e66decc4cedb','874bb70a-f7b7-4941-8faf-884a5d6f95e7','6c946471-150d-4f93-8242-59d0ef74ebdf','828cfbc9-f8fa-4ba4-af5c-3ce809f39437','8b05ee3e-78eb-4606-bfa3-8a5ad11bfbf2','41445e42-5a81-4cb6-9d13-397d61fb15bb','d6e2998b-ef46-45f2-a06d-6c9b8a6fc668','3b445be7-2aa0-41f0-bc69-90fe9ffbed7c','e4aaf89f-5e65-48ab-b766-124a32738795','26a67cae-c340-45da-a74b-da1affb267f0','42c8620f-d529-4ac2-b5cc-32314b8b421f','26fed8a1-b9b1-4455-9349-67a61fd4b8e2','f013eec4-dc39-4ba7-94ee-6cf3f22a5123','e2adc510-81b4-4d2b-bb96-d57a104eca44','84a20c8d-02d5-4b3e-993d-49527e151bc9','bf3994c1-dc14-4a27-9dda-e4acccd57512','25f59fc7-a29f-4d3f-bbdd-b1ed0bf03345','5fe08c84-cc7f-4ce4-8f07-8da792b96d54','d35619c1-3c8d-4100-8d32-175274fcac64','1cfbd450-c944-4e5e-a8fb-0f7682c78cd8','2026f5c9-adc9-4a3f-9278-3c284d6c81e6','6a64c9fc-16d2-4b44-9855-44ba010bd7ea','eb763105-2989-4375-ac88-bdf7e8c668eb','cb1bb644-9ecc-422b-a1e3-b57fa60f21ba','8165eb5e-9396-4b45-b967-af8a697abbd2','725f2f52-847c-4044-8ab8-5e30798cb9df','73c545e2-b0d8-4162-bd03-4ffbef0ef9ab','cccf0789-85ea-419b-b355-21f59219e160','759d9e5b-2bfc-479e-9a45-30c965d2b493','2688d94e-a1f7-4cee-a359-47c430c45cb7','bd768967-172f-4c1b-b2c2-4f19c8b9d62d','50d7d034-5cec-418c-b37c-15c386bbb2d6','ed200c8d-f91b-4acf-a5ec-9ef82d7be74c','72cda01d-60f1-4a05-a121-391d95beb637','d69955b8-7217-481c-ad6b-27bd0906623f','a8faf7e9-4d81-45df-a0d4-7a0422f45d9f','fe3acdc2-d89b-4813-a8cf-1b8c4cea60b2','444cb21c-f4b8-4e23-8d10-ddb8c35d2387','09ba848c-c669-437f-8c6d-9e34846fecf7','948b7047-efd1-4104-aac9-7c4caf929992','3d5fca6e-1d61-4784-ac42-5576a0241a90','b2e03f86-cef7-49a8-a971-b20831b4322e','0ce697eb-aa7a-4759-8d54-b7a4b4dc2da7','a54a3c95-df03-43eb-9db3-8a121074b048','ee6659d6-f48c-4283-bc3e-d45c77f1f8db','64b4eaad-ae8d-42ff-b1d8-e1d060708491','121a31cd-5f76-4b21-a1ea-f21ed0ab6ddd','e5204243-85e2-4d63-b0fc-a6e2d1645d0a','d508d520-504b-4cf0-9bb1-815d1094c513','019d7a33-1e7c-478b-bef6-3a72888a23af','7427e278-f35b-46a4-a25f-912d0c08571b','c15a3561-c0bc-4964-b2ad-a87633963538','81505aad-c03d-4218-a7b7-04c10e901275','42781bb6-a4db-4457-9148-3b15e8f9084f','4cbd627e-55f1-4f5b-8b3b-7e46badfd190','b4bebfa2-c51d-498f-8b30-73b43d2d7555','3e6fa9ca-9f32-4c5d-b54f-6217db804170','7fe187ae-f25e-4831-8a34-a96d1e0f16a9','fa837a2d-0741-4f61-9015-03c1e91b23d5','70f0ed0d-d72b-4091-92eb-f555c7641195','198488fe-73ee-4cc4-a7a5-adca36396a4c','9e4dfa97-149f-46ad-9282-e26c68daef4c','43aa908e-622f-4933-b7e2-d36ef21a5164','0039bd3a-9d50-4ca6-bfc6-1d9f1ce54aa2','7958fd0a-d578-44da-aed1-6ba4a3cbf204','66b3d931-74b5-4fcf-8d91-c3780f23a22b','80bb812c-9981-4099-9285-c88ed3a6e698','8ca847ec-814f-4350-99b9-23966a68397d','9c68f297-bd58-4716-8b82-b97f79c1f85c','953196cb-059f-4191-b71e-c9ee66738fc8','718068f4-ec63-45cf-a9bc-31b476ec1f92','6124bf04-4e09-4b52-b507-1c7412b28c0d','5bce9aff-7f1e-4e89-8113-314e81416649','f996337f-dae4-4b65-bdb4-ff4c9ef694de','5ee9031e-11b7-407e-9ed9-c91841f335d8','c50608ff-7965-4417-a5cb-f592a3f820fb','0bc4fc1f-40ea-4d77-8b2f-3b1c2a4cf2a8','1ab3b65c-8b2b-4b9c-87a4-8596bcea4a41','d6111a1b-1f54-4c31-b3b7-c1dfd07d8d5d','112575a4-cdb7-4407-a45e-39a910c134ae','e19737e5-b6fd-4334-984b-65d9e88c1868','12f6d65f-84bb-4705-892b-4575a3fe22c2','6c6d3ed8-89a6-4304-ad81-01908dc64713','55c18780-a1ff-4fa9-9d87-ede73ef754d0','423202b3-91a3-49a1-adf5-21a591026853','476e78aa-c268-4d40-9fea-26db380d5d50','eaa1149a-918a-4e14-8b5c-afe3d974173a','182a68eb-e735-4dcf-a262-aa92f0fa08dc','9b9879a7-8c81-46ea-a8b0-325124034bc4','c176a76a-91d0-4553-9e15-a59b3d658226','bbdf23a7-f64a-4c72-b2ad-1f97d57556a7','1ae0b7aa-4d7c-414f-9a11-544698971f08','9ab0ff69-3f1e-455c-89a8-bda5dd6d6573','659c894f-febe-45d8-95de-ad71e79cf5f6','12e90003-6307-4287-8033-12494ea7d431','85317ad4-2d8d-4b77-a446-6e6a9181948a','42ed5bfe-f3ed-452d-8b73-7203d2973dc3','ac41a64c-682e-4dc9-a9b1-ef70e305c586','f4223c81-c252-4720-b4c7-41cd793751e1','452b164a-4852-4af2-9e33-abc33fbdf5a1','7047fe1c-a509-4e8d-a4fc-89ddb43406c9','bf929494-0f1e-4dd9-939b-d2f88df1964b','e11d65c7-16c1-4880-aa9b-7c5e4eacbf5a','1070026c-3854-44fc-a841-be8d752a0f94','c1f13d0e-0905-4ee2-ba89-a9d854563d48','41ef5773-0c00-4b13-b5f9-f807b79683c8','6a80713f-0c28-4412-9034-dd2cc3df3e50','feb48aef-13ba-4e60-9e79-047fcd43d27b','51d8147b-a8ce-4674-9144-6178df22e6e1','5acd3c90-ecc3-42f9-8de6-e8d5bb827397','ad05577e-c396-4dd5-ac73-15484d1fa7f1','49b6665d-5675-4d6d-996b-ffabf1538416','6ea091b2-be61-4ff4-9c09-c07b300db65d','72ed0b2a-e030-4a98-a4f9-f04f1c5feb1f','5aff54be-a7b2-4f36-b108-ee38c9cfeb67','e8356edc-e5c3-4a13-ad9a-4c2fc7e5089f','4d4b17f6-a2de-4fea-8819-4da6ec1ebd16','9fbaebc6-0bea-4762-9ece-0233c208aeed','0fe46eab-58ee-4b13-8a16-cc7c092a8bad','03b693bb-32c7-4644-909e-8b226528181a','9d806277-9b85-41c3-91f8-4785d1f0dbb2','8f2e05bc-8ef2-4861-87df-48d08117cac3','5e7b0aaf-285f-4c18-b5d9-84be6f346769','8108a9ed-10f8-4bd6-8cb5-b14d1935429b','6f29469d-bc10-4da0-aded-08e8ad4efdae','01924cd3-44ea-444a-8e8d-54b1883a2e09','251d3387-255c-4bc2-a7a9-faf6a6fdd980','9f49a55f-a74f-4f61-818f-a01fc872adf6','e2071762-8a70-4537-a603-430ef77d4765','3ffcc1de-9cab-4f99-a9c2-544fb1afe522','1fc2ea36-3f3d-4767-b424-4f4389e351d0','0799c2f4-98a7-4cfc-903a-61f15885a222','4174be34-b741-40af-8229-acde569e56fa','be655301-2b44-487e-8ce1-8ef945b48f59','8a70d8c4-3d6f-48a4-be38-cd9044481620','72590f74-dc56-4618-a89b-d1dab5429175','bd3887ee-f938-449c-86e2-b775e789f3e8','490d9807-3538-4a5f-9c41-6a9422b0ba06','e4f7292c-ba01-4926-a402-3d618bb0ba75','fa110eab-5c09-4539-b259-96d6d3eddb9c','4c704dec-4ff6-4ac1-906a-07eb55e178e1','d37e5b50-09db-4448-91fe-caf5a54d92a9','aab9f4eb-c0e5-433e-8bbe-f730f25693d7','aaf250ee-6a4f-4b56-a424-9625e55b474e','490bb849-99d5-4bd7-b925-d73481b7cbfc','62019758-0b7f-4fde-b1fe-e81189918905','13a1df36-a344-45e7-a5cf-a97598c795a1','5731ebb3-86ab-4428-96fa-1d9185450875','4ea8ff8a-3992-4d6e-93f2-b54754ec217c','d40a7645-c10f-4a5d-bf7c-4c4e718d36df','3ea0f27a-403b-4596-bcb3-b9741805d704','36eba73e-6410-4860-b0b6-0e38effa1c6c','25611efb-8ad0-48b1-8fd0-f77136d553f9','2d4d8b66-ec67-4c42-98c5-648ba77159d2','552183cd-e218-479d-ad93-f586cbc1906e','b7a02b8a-e31f-4c03-9ef0-7b03123e2380','e080a31c-5f7e-4351-97ab-0d1faf8cb8c6','853ae931-9c75-4357-a285-e96152905f8a','2e26694e-8e85-4761-92f6-b45e0562a718','6eb599c5-c019-4a53-953a-e09bb469dedb','f1f1d57a-9910-427e-a670-c5a389459903','bb83f6e9-ddcc-4561-b9be-a31193bf0b5b','cb5b9b5f-186a-4307-b53c-5ad0b8a56d44','9d1310b5-a176-4d22-afb6-1262acd30ca3','5a840516-f629-449f-81a1-c53f356eb9b9','ca673d2f-9a05-4cec-8a0a-a14f888faed9','12d1f6b6-13b7-44ba-962f-09b704841527','aac4ce0a-af1a-41dd-b218-7f8d6e65bb5d','8ae6e5df-0bab-472b-987a-a64f459823d9','809dea98-0689-45a9-8ef3-db52d6736933','7070890a-f65f-46c3-a33f-e8b1c34e8577','0521ef7d-aa07-4c9c-9c7a-c063c4efa392','ccfc4230-0c5e-4b7e-a0ef-e39168750624','457402ab-e61d-43c3-a665-6b9eb00fee31','9891458b-551e-48e6-80c5-624608c50d31','7bb88c33-4f00-4b61-8091-4c34863d2305','fa10f0c6-f3c9-4f7a-affe-ca5831c90a5a','22624715-f923-4a93-9cdc-171fdc51cf9e','aac1c944-9cbc-4705-8449-178e0cc283c3','9f74bca9-4373-4d1e-957e-89fbbe81dff6','abc287a7-aa34-4e0a-b4fa-1631ed8b1e91','3c1dd05c-cadf-47f8-8f54-51ce50e4dd8f','014885b0-5773-420b-9b2e-09397141f635','b85040f7-2da9-4fa9-9414-b7e93616d4f4','b209183b-4176-4301-9d6b-a5c4238820d1','ccf620cf-1631-4e76-ba93-8a7bce2b1d45','e0e92bd2-aee2-4460-91c6-e6146118dcdd','f0ca888a-ca72-4366-848f-c3f482f12bf0','e355bbc3-37c5-4dc8-8394-733f223d2695','012d942a-f373-497c-ad55-f8575e278741','afc2a26f-3ee8-4ab5-803e-00d9f211e0d4','c31e422f-9840-4ec4-8609-246ccf35feff','410893a3-6a63-4b63-adb3-97616f5b7e04','a09c5a36-00b3-49db-a96c-dd6c686dcb37','72dd594b-bfa7-4b15-a582-672f73da2b1f','2676e678-1d64-4102-ba4a-689cc7e3ba56','85bf8984-3705-4a6e-94b7-cffa861bf299','2c85b742-2403-49a5-8ada-02903b15bfcf','9de5c64c-a889-40d1-aa2e-41d086dc09d4','70321679-4645-4324-98d4-04c4233c0ade','ab58aa4e-39d5-4b84-90c1-d66cc70e0506','974001b1-bd90-4cd4-9691-62dc4c986e51','d41fb471-5c72-45e9-b4c1-7632ce6c0a09','0abce4e6-7e7b-4591-b225-20d61df58fad','9a60f09b-8961-44cc-a3f4-0df45471d7f8','790056df-f5d7-4045-bade-cb7aa96a1f5c','c9f6b8f8-8dcc-44fc-8031-2a1c0a38b7ae','ecca00c8-5ca9-4b31-abb5-3763df135480','e7a23626-bcaf-4b90-84c0-8641ed20e52c','18ace4ac-b011-47af-901e-b8e2bfaa3690','0fb9a088-ebca-4007-8b2b-aa6c2bbbc121','67065b07-b09b-4e0a-8bab-1e0fb559bb54','e4fe7b26-15a1-4a60-ac88-127eff401269','97b07090-2b1f-487f-80ca-2d81e7471644','7c9cb6a3-03b7-4005-8498-ddf5edf32b1d','0d4b276d-2b0c-4e62-948c-3a6e036636e1','94b27a8a-197b-4ce0-ad2b-c436fe60bfd9','128af02d-76bb-4c8a-8cc7-cf61efa9d980','a774c5ee-7293-4627-a3f5-af44950ea87f','e81e7ab9-0e44-4309-863d-82f1afa93119','8d2412f4-7487-4b9d-9da7-31cbec1c1550','97de4587-9999-4387-9eb0-978c5a64da08','e8df6000-652d-4992-90c7-633813b9eff4','f542215f-0644-4de7-bcdc-bb1603fa9b8c','a5504dbc-c3c1-4dec-8225-79ac56cbe8b5','0e823eb4-5f2e-4e42-b3f1-90d47648b7e4','4bd47667-9bb9-434c-a0c5-c859d5131123','6e98d8ca-ba9f-4800-b25d-ae435a9efa39','83ea2612-1413-4c98-b535-49b555da2565','2b621864-f5b0-40c5-ac9a-c2a6a2056776','d262533e-988f-4efd-a1af-64a36ed49ca0','3c0aebb4-ced0-4a99-b140-3188b18490b0','959429f8-5d50-45b2-a4d5-1e5453fd2bd3','cabaf953-3e32-48df-8cde-1fc51b511a18','56ad54f5-4f8d-4b86-8fc6-76522985f462','c13fcb6d-cd7d-44ed-8d76-8eff9449f4ff','0957ffea-2d7a-4937-9539-4bc3a182b6a5','2a01a85e-5c59-494d-86a2-da714db0bf31','64b6baca-4ee1-4060-9a4b-ab21d6ec09f5','a677bd4d-9140-4856-baf9-1662e7994539','6fe88e89-cdbb-4855-88a4-88d16d827e81','2ca2e85c-d2f0-470c-bf1f-d0bc350ed9d2','ce2c9cc4-d07c-4e27-856b-912be0408029','0a493c79-1eb7-4c71-b032-f445b01904b5','625e964e-ffc5-4ccc-b771-dd1ec71dde87','e9f3c633-1a41-4fdf-834e-9869d40158cf','479bee72-4765-4d00-ba84-571ab8161116','c0530267-6e7d-42a5-adfa-75b1e59adeaa','e7f561d9-ac04-4c9a-a1d0-1d550e856675','e3812a29-881a-48fd-9c5a-9a1f7565bec9','af35f88d-7c89-4546-ba81-d0c6e641f2a2','f1580adc-cc5a-4058-b348-692a4f51d7f9','23a0de56-1806-4448-992b-c8c4982d1551','0746d51e-3344-498e-aa76-52f05b26d6b2','e80d0945-d4dd-4ff6-81c6-1c3a14031f58','554c92ab-eff9-4153-a23a-1d4638d17b34','93982d9e-a18e-4137-947a-a986903dc0ca','8f33b379-6e15-4409-ae77-93752575f0ae','c3593552-d654-4f88-9d90-f5e4efac1685','84b2df1c-b143-408b-b184-1a98b2b60199','46e64731-fef9-4315-b7c2-add03af1875a','3fa48bd5-6928-40be-8dec-7d8ff614e244','9848e5fb-2797-4cfe-807d-4d0e77f0b12e','e9c3cad4-9e15-45cc-a19a-5c6607b26939','e9bfd96f-4822-452e-94b8-b85105e6bc31','eac2e2b5-e38b-4833-9cee-6c87f9a18123','f6482607-304f-4bb1-9687-657675386ac0','ffb953c0-d818-4688-8bdb-68d4f44dbf32','addaedb7-e53a-4884-ad20-593c88c0c257','713af5f3-7978-40f8-a26f-c95f90e30be8','40d3d66e-f43d-419e-ad60-bd8a6f633c53','da25b4e7-7d48-4402-abec-308569116908','e5bd1917-02a9-41d8-bae7-d6dae64b8a11','3d434d02-8672-4df5-8a81-d6607d2e853d','7708e553-2595-49ce-9d88-4ac428db8110','b52cc845-0302-419f-9ced-09cb4fa2728d','f7aa5e69-5137-43f1-9618-21153f4c2ef8','bc6d4131-2ccb-4597-aba4-8ec60fc34682','dbbf6e8f-987e-44a8-8123-95edd624b680','f12b2c80-a91c-46f4-8e02-5173a83dd916','1fa8575f-02e6-4943-8117-c3f9f3595270','1ef3f046-3b12-4b14-8262-0414a44c41fe','ee391016-623a-45d4-9e67-3935fc1f924a','732482e8-eccf-4115-97e0-f81b675fb953','7289faf2-f986-4908-99bf-cb2679ae474a','d46be81b-6213-4ebf-b26b-c1ad64a3bb6c','93e17827-020f-4840-b48c-ba1b364237f3','93834b1e-88f7-48c7-91eb-c21426a5fae0','a47fc7a4-5a2f-480c-b4d2-a3107068233a','9c5296f0-c2c6-4382-89e7-427de7efd8e3','2b447124-c977-4a08-a087-41100d1c3e47','fed6ad38-380b-4f9a-9ef0-786855c8623b','38c5b515-fd68-4f17-a4db-8ae334be6afc','ed6f81d2-da7e-4062-9aad-0474cc51ab0a','ed06dd80-426e-4f84-8d7f-0f55408d4012','cffe62f5-09c1-492f-a359-97d0dd498999','b2bcc0f0-91cb-4ab5-bd4e-6e9fed7a3596','653d1c58-1e2c-4c6e-b647-2fb099af0ce2','d22f2352-00e4-4791-9d91-83544c70550f','b0d328b3-7ae1-4b5b-9875-d085849a2e7a','ca8214ad-c61d-47f7-9af7-dcff565e9e32','96f78945-8913-4d46-8638-cea3cdeb99be','1d95f7ad-afed-483f-81f1-86fa0ae247b5','0ded3f6a-b421-46a4-876b-8f3bdce12f27','b47a39ba-7a97-47ea-af25-03b8085184a3','a78f789d-0ddf-4d1e-89e0-773b8e2dad57','f76f5949-ddad-47b6-bdd2-894c29bbb55d','784ceb2c-0b14-42a8-85aa-99959ef4a048','a214077d-d324-4105-b43f-2ba945d2d436','4236aca7-159b-4c44-aa2b-0e072e14cec5','71c1c9cd-fbe2-4b42-a68b-359d0545c672','420a4c7a-5e56-4f34-b9ea-7802ac23961c','305ad787-5a4f-40cd-b125-177009cc6111','ff06f955-4083-40f7-b0e0-ef08c4759929','d25aa17e-42f9-415c-91ed-4bc6dcafb350','748661d3-38fe-4500-aa5f-d4584589fb53','50d8a077-2926-4243-b86d-1a18941c38b4','a02c2c94-a5fd-46d4-955d-114b5d6190da','bfbecbc2-f5ac-4007-9f2d-2f9f867e2fab','1f3aaa28-67a7-4e1e-a1c6-bd4d7cb73847','00cd57e7-46c0-4bee-b1d4-f92d5297f337','d9945237-e044-4605-bd24-291d215e4a29','9aa168de-dee3-4753-bbf9-c46a9690218a','88a44795-39ee-4830-b69b-21397989dfe2','c1b9b2d5-32b2-45fb-a677-ccd9b472f919','0961db82-e35f-4e37-8500-7bc278c7132f','d49eebcc-aed2-4f4b-a438-54af8a5abc26','49a6d4be-7c5d-473b-aedc-f0f9f65fa77b','89a8c5ec-1bcc-4110-8410-99357350a62b','6e48cd24-a2f7-4a9c-bb96-c95ab8619f64','5393814b-12c8-4942-b69d-79df35302acb','c169ad36-5455-4db0-b768-65a54d1f0d1a','07035a77-5e0b-4214-89bd-f1b2f0ee4dbd','08ab9cb5-0252-4170-b56f-68e18c4c5409','7e8cf8a0-da0f-480d-ad81-f64ee4c88668','cf67dbe0-6adc-4279-9865-265832754496','c25cdbdf-03de-4add-90f3-8bcec00ae300','170c9c6f-8189-4961-9f8a-738f197e4dd0','58eeb3bb-4b73-42af-9a7d-4dd8d8bb1cfe','54d9fd2b-e61f-40e0-8463-e8e0f2b31c86','b0593ac7-df7c-4127-a515-990dcfc574cb','4e326d9a-4e98-4fef-a3ab-91ac7dc58371','8aedfa62-a0ef-49ea-ac5d-22149ee72cd6','29b18905-a6e2-4a05-bdfc-b2b9df1931fd','90de7563-e9e8-44a3-9614-b188910d79ea','bba5b51d-75fb-4a6e-8f4f-4613af6dde77','d261ed0a-f75a-4702-aac0-8860ad2af321','6ad800c8-3cbf-4d3b-adc8-0c3811eea1a8','5af647b8-18f0-42bf-b558-6364b50c5027','79acc337-9316-4192-9670-9b5ff0348b04','4d8e4f08-ed27-4dab-906b-e2be553819b0','6c75f0e6-4b1a-4b70-9897-15cc9e69c996','40e132ac-0121-43b9-ac90-47acd93afc9b','f954318f-a150-4b4c-aa1f-67208387b177','21d46dba-aee7-4242-b44d-d39b70ae287d','d1868b0e-479d-4d73-8947-d70b3ca645e5','7bff2eb5-5788-4853-aa79-c38a7eac50fd','b8cb684d-d0ce-40d4-9926-fd3d1fb9a0f2','baaa3ffe-352c-4498-9357-b7757aa08ed2','50e9b5f6-3860-4da2-a9f3-ab19c4fe4a85','ed450422-3798-4564-a653-deea569bacdd','1fd96648-cf23-4fd3-a90d-47c79cc8ecee','547f861d-3bbb-4c1c-a66e-9cf0217a5fb0','b4462e03-a86e-4060-80f6-ff43dc0c4fdb','5205b826-2e79-40e5-b0a5-8f2f0bceecf7','f255f0f5-be25-49d8-86c0-49ce25d66d1f','fb3d1897-3cfc-4705-9a21-fd58210f7154','d05abb8b-d3fb-4e3a-bea4-0e68dccd20bc','273e0433-0587-4d54-8846-41827071c5b6','2a70c006-8e1f-4503-94cc-81931204648f','6141c95c-3745-4882-af8b-6083b5305339','c86ff87a-c00c-468a-9ad5-a5c6a2e947ee','b30d7eb5-71d9-4a90-82de-2bda6c9f1d5e','933f2193-b162-42a4-ba0a-7e1641bf7378','bacdb7d5-69ad-46a7-9103-7bc89be47a42','4515dcd0-213e-4021-b6ab-c373b0a5b011','1537fc1e-d4b0-4ea7-b691-abe4ff5e9815','e845c2e7-ad7a-4f8d-a72b-841d9619332a','3e199577-ac68-42d6-bbf3-27677b2ceecf','150ddf65-74d6-4b86-8e4e-f6c9f5ace76f','111c8bfc-5c8a-4b14-b119-cb50e49bd1ea','5b1229e1-d9b2-4264-8623-86034d0e4633','8c77a9c8-7045-4a38-8f4a-fd3b135963de','d667abcd-70ad-4fee-bbcc-a51219a9993b','85bcd796-df74-4991-803f-68c33906091e','c4793d83-1284-4d43-ad42-31f18115fc16','940f9bd6-4da1-4a48-835a-c7e39f09a3e4','8a40d735-7149-48a2-8b78-3126b873460d','e5746329-3fdd-48e5-96a1-20fc71fb40b1','b97e88f5-93ca-4350-b2dd-62744eddba6b','30499d24-f708-4b92-b5ad-83349a29797e','d144c2c9-93df-4e8f-b1a0-feadaf2f55c0','399f400a-d406-4ac3-80d2-20e08de39914','a1578c70-3bfd-4727-8c75-a8c1986c391c','ff7abc78-daad-47bf-9232-99397582f0ad','9f6228fb-f12e-4e5a-ac50-7715a7bd7d78','b907ecad-6699-4b8d-a63c-4ccab98d5a32','f4666ff7-6401-416b-9fc8-8c29f6d3dfa0','73bd6aaf-439e-4885-848e-e88bb9071c93','427da588-2c3b-417d-9da5-8e3f19346861','5bb7733b-dc3e-48c2-a7fe-2ed4176e78f2','13c951cf-9481-44db-b679-62d9c772270c','c47a7a03-b0f9-43e1-8bed-759cb89604c2','275a93c6-7ba7-49ae-94b2-a1cfadc44371','6f83550a-0782-45cb-b643-7112c1fcfc93','b33e3256-124c-4f5e-82f6-8fba72436327','9b044bd9-f7dc-4049-937d-b042f14d9b58','690c32df-0fdb-4619-a4f1-7f6003547fac','ea3d0940-1b2e-44e1-8fc9-c7f2049b99cb','dc74f852-8fda-4560-90a4-2cae6383f43c','06cd4058-2932-40c6-9723-13e88a5639b0','70920c19-baa6-4794-bdfc-161e7c73c0cb','8810f613-ab75-4f1b-b2b6-8fb821de6783','f92e1273-750a-4333-8569-101008e15d52','b461c576-e6c2-4db7-9eb6-3db283ed428a','ca7faf3d-1075-4997-b432-cf7a3b3c2b59','0bde93a8-a4a8-4ac6-881f-c61d52a7bd7c','56f18bd7-3a10-487d-9120-de9a416c75e2','394cf4b7-7e26-498c-a6d9-1c313c0ee61a','bcc452e8-8a39-4de1-bdee-639435d81adb','fb4732b0-b9d6-4af4-ba0a-c68354f72152','4a725e4f-e5bc-4e4c-9b1c-1664743a5cc8','176aaf95-f74a-441f-960b-678252595a8c','e5b0a49c-e847-4084-a2f4-5130f32458f8','ba304ed3-e5d5-4118-abd7-847580156eed','43ac3013-fad4-4681-97e6-22940958a07b','e329568d-0bfe-4a15-b93e-eea44f6310ef','f54c53dc-b06d-437c-b647-a79bc69de31b','aa5d781d-f2d9-4cef-aeda-3b4de90d5d5f','e86d7f54-80ad-47ce-afcd-90edbcb1c3ac','325798b7-e40a-4df4-b279-9ff81d796e29','811eed0d-cc4f-43d5-8658-1441b7dfb9f0','ea0b3c28-51cd-4815-a39e-8e9abfbe5cec','3bed5de1-1c3d-4ef6-85ca-353245e51ec3','d85dba2f-557e-4df9-ae56-a8bd4dd083b1','ed7170a5-a616-4eb1-a929-ecf7d1cec488','d7ab2e60-1548-4c3d-93c4-3c5285294efe','e6a875cf-57af-4b14-b8fe-0955392f7427','0a9ac267-7193-47ce-bbd7-a988556dabe5','fe3375da-870c-4aad-a330-eb0a2644f8cb','c88b40d0-2d1c-486d-b11a-aab725a9f64b','c85f219e-3fe6-4afa-8fc9-ae04b312b0a3','a1d19051-2da3-4e8f-bc67-24d829a1a804','d7e6daea-1e2f-49a9-94e7-f5a14c847200','36c771e1-6aab-4a91-8ed3-6522c8e98c26','c7c648d8-ad4e-4a2b-956c-e5561a1d31c2','c7e2b4fa-f6e1-48b7-ac34-8ccee9b37c98','e5121fdd-a403-48d0-9a9d-6d1cd855441c','1f1d3bfc-07d5-41b9-88b0-ae9185d3ff01','6f5d9f50-09b1-4d5f-96ca-d92bbbf2106b','ac18c84b-52e9-4ac2-a7c5-29ab295bdbba','4cf131dd-7a0a-4133-ba11-6606b46216f4','9f6a3b73-ecf0-4e51-8d7b-2384aff3616e','d4aa5ac2-d9b3-4a20-8051-f63c548df448','b36637d1-c1a6-42e2-bc9a-970abc3325f0','e50423ee-d3e7-4204-bc53-4f94a80aa5d3','a413acd9-de0a-4648-b980-a913e835ff8f','7c7430c4-cdb6-4ebe-8cb6-f794df3a31cc','57997b2d-5129-42fa-b6f2-00eb906e21f4','41f1f1b5-8370-46d6-a678-93b5944a6502','1e003937-5060-49f3-90c2-62ffeffbf133','77e3bb69-911c-4c0a-9532-d1f4ed14df8c','5e6ac34d-2850-4399-b170-7cd15831c1e5','7f33d46a-23a0-4cf3-9956-601de46ec220','fb050b4a-18e3-44cc-8fc4-ff8da7e3a4d4','ab002446-b9b3-4d08-915b-1f5129848b36','225321b9-aa62-41fa-939e-71f5ba831f0a','81d238dd-3dc4-4703-b793-03f66258c7d0','a3af9878-fc79-4df1-9f0f-65975e6573bd','f664259d-01c1-4309-8f9c-3b0c2d80e818','4eb7a799-b0f1-42e9-ad2d-7d27621a418e','08362f06-ec3a-4d78-b1b6-4198dbce002d','87d7ad26-298f-4565-a72f-82bcad1a19e2','a7bb513e-1b10-4eb5-b0c5-3f97006dccc5','405a5473-15fc-444c-806d-cb32e9c9baf5','fb29d636-cc67-48f3-9b34-7c740bd9da11','0d347071-5d60-4aea-87a5-5576fb90e88f','3f184d70-69a6-4b7d-ae68-2cc34841c83f','4907a4cf-c3e4-461d-92ad-e2cee1d75911','f5f2989a-cc71-4737-936e-4b091eb0706c','aaf89080-a2f1-4e2d-9c03-bbe511d1ccb8','956e048f-bdcc-4419-96e1-c551c2dada33','4c34e83a-0980-48be-ac2b-ae3b6d78f9a7','f78a26ee-0d6d-458e-9c48-3b035393de0f','876ecb34-0467-47f4-a703-ab2ebda4fba1','f5fce2a3-af6a-48e3-81d6-5ac604bb94ca','0d48cba0-34f2-4d95-947e-321c5509c067','af089692-b089-4706-9602-900e83246eac','4e73698c-b08d-43f4-b6fa-8a8626509f97','c66a43c8-cd99-4160-8386-3d33d7cdc854','3bed167d-4a70-4912-9d73-7f269d7867c5','a37dd7a6-dece-4e70-a9be-76834322733c','d3b81e61-61b9-40f6-8e7e-316c0565c354','07a8f166-e1b2-4099-96c1-5492979cb7bf','8e725d32-f93f-46ca-af38-c42970a19875','3833f7f4-0246-4bd8-a054-b301eafd7aa9','e672bd4c-c128-4cc3-a279-a30e2c9fa35d','2df0c462-0aad-437d-8cd7-bf7e42c6c83c','0b6de99d-b099-44ac-aac2-a008bce407f1','b3c25895-11e5-436b-af37-6f6a6819707c','19f4b52b-0900-4d19-9316-1e480dfce5ab','1ae84b14-1328-4f69-9dd8-2d4c672f950f','c00411a1-bc0c-4444-ae5d-39ec491bd801','88211d5a-33ca-44cd-8ee7-6f6f1445001b','bacfb651-f3d1-4b71-8318-879997cce961','a3109b8c-9e70-410b-8d15-413ce75b613a','68fa8882-3301-4dca-92ad-b1d3ce6bfc1a','31f61860-616c-4c3c-a3bb-38a26d9e53cf','b4b9ffb6-a884-45fc-a740-fbb0c7975747','82e8620b-30e3-40b5-8a16-d4b28c7f5656','77a4ee44-fc61-49a4-a070-862d52fc343a','0c0a60f3-124b-4440-9ded-73152bb02e1c','94b55e7c-526e-4cb3-b886-f5ca015571e3','b3f65b22-1eb0-47e5-a43f-d5d8b4050934','f5ce4726-5ad5-4ef8-ba0a-72b95c9470fc','d324a168-83f9-4217-ae1e-ba3d22e450f4','2bd590eb-7ac5-4982-9f71-a58981e7fe44','3af47880-8e33-44d6-9585-fd064410d001','499ec051-ed5b-454a-bafb-e70115ca530c','56199144-2cfd-4ed1-a7b5-df742c0f3194','0eee8a6b-06ac-46d8-8b29-617c1a3e6b94','209a23c1-2b47-47a5-a890-20ee0150e502','bb39139c-09d3-4f69-8a7d-eb6204f6a091','4b3a5bb8-7012-4c5d-b496-3ff142985e01','2fc3f6b7-089e-43cb-a3b8-fb52c74af204','96b27e30-5e3a-48d4-9e52-837f76380ede','e49b07f5-7483-48ed-a566-993eaeae8098','37c17522-a526-46cc-9ae4-5e3aa8b7edf3','90bf88fc-ee5b-403b-939c-66a91f25c65c','709b672a-c90a-434a-b0af-128e55f8b11c','1f3ca79e-3710-4a8e-936b-d5857971152f','4759c480-bf47-4109-941f-6e6e6c5372ce','ca0a8250-babb-4c3f-8b80-3566e5be1a19','2b695764-04e0-4388-8264-0e52e974f7b4','310866e3-a708-4dd6-b2df-3f22f6846440','22bf28de-80d1-4137-9f5f-0a53f9efc905','e24f575f-eb24-4d7d-bc35-4f617f038a75','541794fd-3f0a-4298-b7c5-16dda73935ff','28728481-7688-49ff-9948-bd52fd6fe5cd','7cfd7730-eb32-4b25-b099-249f5a0e959e','e014559f-5d2a-4cb6-a567-3f95b84369c3','262bee2e-4bb6-4765-a1b4-efecca8d5237','f29e6983-2edd-4a78-94f0-e91dc54297c3','0bdea338-faac-4fe5-9f7c-5481ae5735ed','81bfc948-4439-4d24-889a-19ed9245d9eb','c646ef8f-361e-4e51-87bb-2eb7837abdc3','6eaa6c33-5587-4073-8870-afdfacb4c5b3','3b7cc31c-7c57-461e-924c-eb9129490aa8','654528c3-8eb6-4e22-bb00-4cf80135b4da','bdb2069b-b3de-480b-8ce0-1d79edacf233','3b907c66-620a-4441-8277-e8b521bfd121','bf1d33aa-c129-4e68-a054-fa75bfba2e61','aa4576d5-6f5c-4697-bcdd-1db6a71d843e','0f2d4f10-adaa-49bc-a275-96bba41a01f5','ee373b43-945f-47dd-837c-d1e27697c703','2bc2c490-70fe-48ac-b1fa-056ba23625d1','fb7a7bfb-f378-48c8-bedf-1a33d3684a45','ea6e2deb-5e28-4ef9-ae26-cb5142862a26','90906e16-0921-4301-a3bc-bc75fba16f81','4186a552-4a10-4f85-a5c6-beeefb88956d','dbaccf47-988c-440d-97a7-a5cff41b344e','34213a04-2620-42cc-b4fa-ef8921c23cf6','9447a68f-aa9a-4d9d-94db-5fb2a190ac95','fa46cf11-5a51-4927-b3cf-c8e06241f43a','77978586-287b-4753-a8e8-6276a24baf2f','ac1b78b6-e917-4b79-9631-7815aa862d4f','88b475fa-7752-4259-b59f-2b372b74bba6','cf2628d8-31fc-4cda-84be-2ab12b0f77fa','c9d409c0-9348-4a95-836f-fd67e244d4b7','68f02c71-096c-4c3c-b3f7-40fba309f594','4410ad93-38a6-4c00-8525-9457e5ed8ab6','6140f104-84b0-41a4-b766-f5eeb8e28ae7','f45b2e6e-9f9a-4821-a805-1b1da372bb39','95aa82d4-8e77-4959-aea4-6cf7d2a93745','892807e8-437e-4dc8-a4fd-213b42fa6452','c2a34cb0-a8ff-409e-9951-20018a3fe098','531b2503-6d44-410f-a8f5-ecd727592c1f','22d0215c-9076-4a4e-b178-83acfd9ef613','83bc37fb-48f1-463f-bed8-ae4b07db97ce','c6f5eb2e-1fa2-4b88-81a1-2c13f3d821b2','2ca32c79-cbb8-41eb-af51-ea9958a40396','5ab19e3a-5316-4e37-bd18-d54a08f726d4','2a325eaf-5c60-4dca-87a2-0f7cc55de6c8','7cb518c5-8696-47b9-85cd-ad66fa2cb4d4','2992885d-2f28-40db-a5be-a50f1fb89060','1681bdf8-d3fc-486d-940a-2022374188cd','9c868d58-975a-4eac-b237-70d30e818a7f','426e82c4-2458-40ed-a0e4-f9ed0ff78e1d','f10aacc8-6ac5-46c9-a6b4-a308594d3316','5afd2bfa-c76e-4a6a-a0da-693e3080da0d','bb5527f8-5e1c-4e39-8581-db1a1f5e5be1','6c09b6de-c182-426c-9d4e-9e6e86449d9c','a1aa84d7-2751-4150-905f-e77543ea6913','e849412a-3019-4a67-a480-460e34758db6','82fc7ce3-7f3b-4203-8ae4-a559259f7e35','82159097-3ab8-49b7-a8e4-7d52d2cad0d5','2c1321a4-15f4-4af6-a5d0-5502ba31d38f','a444a717-2ed5-40a2-a8d8-b6e3509c15e4','876371a1-4f20-4a44-b1bd-55201f2d197c','2d3afb63-a715-4422-a191-20461ea529cf','2624abd8-9c71-4c9d-8fc7-8ebe251cd1ea','121fe815-62b1-4be5-a635-230915ad4fcf','3fd62765-491b-4563-bfd7-d8370188cded','8fb4f7dd-ca54-48f9-91f7-d5e496b3a565','610bcf43-ae1b-4815-9647-2d38a4cc52cb','05f09373-91d4-430d-92d3-819a2ca2c83a','76f1ee03-bac1-43b8-a147-80c90c4d629f','42bfcb1c-e799-495c-8044-96789406cf77','0a278973-5d80-4095-a052-e44de40345a2','6802e9f8-aeb0-4730-b918-09389e283302','149c369e-e257-481a-9901-9933f7d9fb97','aab3d3e2-e72a-422e-ac58-7f6811830676','cf7d43e7-a7f2-48fc-a0b9-ac65923f96b4','4824a3c9-787a-40b3-9f32-169ca129058e','1b27b651-455e-441e-8a33-3b67a338b8b7','eb0095ff-15c8-4f5a-a498-077301daa797','41584cee-f7aa-44dd-914b-7465fb788e78','3adcfd50-45e2-42e9-8ee6-d4a1cdb3b1b0','fa4ebfc0-2506-4583-9f6a-0aed092fd72e','508c04cd-6b60-4561-9bfd-0f76c8fcd220','1272a914-2694-4d80-bd19-f84e427ff0b9','b8da2baa-1a67-473d-9df2-1ffe97322842','d257c804-fe5c-485b-9515-34bc643aa179','659925ae-bd2c-452b-8de8-5040ac12a7e3','5f86bb3a-390f-474d-a8e7-e7fc09f982b1','04702ddf-247f-4039-9b0d-cfe8aa9ebf61','224e7474-1332-4fe8-8d20-9bc0128170e4','9aeccb34-f284-40fc-807a-5a03bdaa1097','1ad4e146-b693-4c04-9c67-01394a297c1c','1c759477-ad92-4bed-81fb-ffd1fdeffa91','e9d4b9e6-a83c-41d9-8e51-9d9976ce2fb8','876a963e-123e-4979-a2e1-a3c2f355f4ea','f6343412-6dc2-4ec3-946c-13656a6a1e13','87013ef9-172d-44c6-ac32-7d404587ac81','f369fdbc-39e6-4058-b07f-292a04c12c77','51191237-3a5b-4583-9dfa-46a269e365f9','f07364e4-353f-48ed-b4d1-6170cf9558c7','97e69a97-d813-445a-8f3d-244066edeefc','6221eece-5633-4aea-a752-fc3e3226f964','98636875-ee82-4efa-9bbf-8517e47d61e3','8500c7bb-7a49-476c-a434-1603e191feb5','4eb62ded-6ade-47cb-bd86-0486bf57e984','280c4c8e-6eec-4e93-9dfe-3f677dd18849','5d5c73a0-8635-4d30-b1f0-730d9507322c','091b453d-b35a-4e76-b1ab-b046d9eeb9d1','a263c5e4-973a-404c-aecd-9e08b2c06e76','205e4ef3-2fc2-411d-9082-f9cf46e0ba08','b6469852-5b8c-4455-aca8-3150eec12ea2','8a1b4dd4-ff57-4995-bf0b-c0676a3ff742','2712d62e-7f9b-461d-8d6f-8dd8d09feb71','6141bed8-9653-4c12-9747-385f60e44894','480a8c19-2a1b-4771-b079-b4674a297cb4','fae02e05-fc94-41ad-afe9-abb8773e7185','3c1c78a0-7b71-4aaa-8aa6-7b5a0f4ad656','8a2983c3-2814-46fb-8156-ae95829bbe9c','350b15af-e122-49bb-9b9c-fb695dfac05f','f5866ca9-d708-4711-82c9-cef76e946a8c'}}),'113656',struct('BlockId','eae6f9ba-ae76-46ce-93aa-c1a394602c66','SignalIds',{{'80c2204b-4dea-4de9-b596-4d15d491e727','6ea81466-c3d0-4102-9e67-518f34ca9d65','c34f03c4-72d4-4029-87dd-b6c9f4add09a','ed077cd1-937f-4904-b46a-7c7ed3f9c927','e9cd0357-761f-4fe0-97bb-7d411a1b8020','25046cd0-ad8c-4ca1-bd28-69946017673d','b3a799f0-4cfc-4fcd-8e32-d5946c1ab4a7','a0ca26c3-c05e-405d-8f46-c053b9edfd30','bdcedbb0-33c0-40be-9306-9dd09256dbd0','eb630ecd-5ec1-432f-aec6-46e4396fcc6f','d2acab7f-85e0-4f4e-92f8-39023bb137f8','ffa6e5fc-591b-421c-8a54-1ce787615da9','8824ad6b-1c00-4d6e-9dca-ca0aeeb7e771','d8b746e4-908c-497d-9458-53b8b3f89443','5de1d022-cd2d-46f7-9706-50a53106b4eb','62f98e70-7425-4a13-b28b-e78f0af01178','3d09a49e-aefa-4d06-bd51-a8aced56b021','98b823c5-9acd-46e8-ba95-8b460a9cf48f','f0b74c7f-70c8-4969-9398-b5955f481d67','70f1c939-bf26-411d-b712-86c3eb73fcec','5a43384d-4952-4b2e-9cda-ecbaa9378abb','a558def1-cbf2-4ec9-8c50-8daaf1c3e030','4bc689df-9bb5-48ff-8906-571c82a13b85','a5baa65b-e062-4d45-bf21-a016c5ddc9c8','099c04cd-e5ee-47f9-a3a3-ef037d3cd076','7059cb3a-d090-4a5c-bde0-3228e8d040d1','33cb5460-d217-4b0e-81c9-d17e70dd7ba4','cb7fa2c8-76d4-4360-a572-e2e9f885c14b','5e6e2242-522c-4593-8924-0bd0c7821f6a','bc49ee11-9f60-4d03-916a-f709ad079014','fe6f8316-23bf-403b-8f5e-baa651dc421e','c7157b82-94f0-411b-9b51-9206b45ba514','779cf9ac-b568-46da-b04b-a177ef0d23cc','fe24fe77-210b-4228-943f-78bb317735d7','edd42d43-efcb-4c9a-a30c-4ae7fb1e273a','40b6e06a-c0dd-4428-9f51-3f64526bf3e1','d7f84817-01e3-44ed-baeb-4af39f31bd1c','23f234e9-43fb-4faa-ae36-4e096747f185','e68f76fb-0266-4186-b9be-bf6693f476f7','e273a2af-640f-45e1-b6cd-2b2172da58d5','679fe4cf-55f7-462b-8166-7dfa68a1dc43','a5d5fd97-c677-4406-8440-60446841703c','5b6f0d52-3d5b-4791-a4cb-8eef82edb229','02258467-0ebb-43fb-bb71-8ea9d5a41328','c56f0c72-8a0f-43a3-8dc2-fadc98d26488','e4080b13-8f73-48df-8354-7b6f3a8b9bd8','dceae4f9-eca3-4881-b313-a63eb8904476','052dabd6-757b-4db6-a03d-6d30d2faa688','6d951047-9ef7-4af2-bc4c-038d732d8daf','e924cc00-b53e-4d9f-9e92-6b2d34ae1f2c','3c3ff4a3-4c21-4e32-9300-f90234613fc6','8a6c66b6-d908-47d9-8727-d52373fcc1e2','fbbc827b-954b-4399-8dfb-7f876a724bfc','f973befd-5eda-474d-a43f-eb31968f31b1','c1beef20-629e-42b9-bc76-807bfbaa8db0','9a1cf17c-349e-4799-9a04-63671842da13','9145bdf5-1863-41f8-ac70-792bb16fe9d0','57fe648b-6999-43d8-9af5-46fdb8ce5c83','60b237ac-89c4-4ced-b2c1-f448e977eeea'}}),'21535',struct('BlockId','2585067a-bea5-4000-9f4a-5d4a5318ba82','SignalIds',{{'61f4e782-3c5c-4d26-b38e-7ab3a332c17d'}}),'21547',struct('BlockId','85c6324c-04f2-4bb9-ae49-a2215b872cec','SignalIds',{{'0e3885c9-c264-45e6-aecd-762fe1b73c31','1baabd13-ee21-4652-b6d4-ec6abbd58849','7652d1e7-3cbe-41d8-a4c1-1dd8e2fc5cb9','7bbccffc-d9cf-471f-ab9a-2a8c4994da51','a802a3dd-5a68-49d5-873f-4e8d27fb760e'}}),'27021',struct('BlockId','bdf40dee-effa-4f83-9fca-9a80da5144bc','SignalIds',{{'6c1ed526-1be2-4bbd-bcae-90132b9ce65e'}}),'92362',struct('BlockId','5f2025b8-49c9-4174-a50f-9954f6fd5e3f','SignalIds',{{'62732959-251f-48bc-bb75-6563641d8800'}}),'92364',struct('BlockId','c5b5a8a9-c0ca-448c-8db6-cd3c9b66be1d','SignalIds',{{'6344fcee-de29-4e13-9955-19d1b344181b'}}),'92365',struct('BlockId','3ece8d90-f93a-46f0-9ab2-53960762ed99','SignalIds',{{'cfb6b582-641a-4870-88e5-47bb370f67ba'}}),'92370',struct('BlockId','1d9a14ab-e7c8-4f8e-b2bf-038c92befc3d','SignalIds',{{'b73568e7-b091-4dc3-8ca8-153143d1aab5'}}),'92371',struct('BlockId','7fa2fef5-94db-4989-85dd-77beb36f0834','SignalIds',{{'1dfec191-1e97-447c-b39d-1186a18f1d1e'}}),'92380',struct('BlockId','e7881de2-179c-41cf-9bdb-b87de17e3ea7','SignalIds',{{'d99500de-b16d-4559-bd0e-e6dac15a0288'}}),'92381',struct('BlockId','8780eea0-5b4b-4d3e-83b3-1728cc0b02e5','SignalIds',{{'20014170-9a8b-46d7-8859-1368f7d75241'}}),'92382',struct('BlockId','29917c35-f334-4b7e-af81-65afbf6f4cf5','SignalIds',{{'984ba9ee-211e-4012-8798-bcbe500a525d'}}),'92418',struct('BlockId','c5a7be29-3173-4b9a-a890-b4cee331cb8b','SignalIds',{{'79a90cdf-8a9b-4ccd-8944-69c4469088c1','35cd3c97-8160-4258-a864-27af0ad45a59','a068c4ce-1004-4dff-b2ee-cba0a0b81dfe','05630d0b-4185-49b8-8feb-e160bf4c7342','87327782-42c8-4aa9-829d-57e10c6a236a','32ec414f-0201-452a-a464-db511b140477','a447bd14-b398-4e67-a61e-10660811da2c','bec63126-1009-4953-9712-db8f6ef516ed','b2eff86a-b6d9-46cc-97fb-d1becbbdd2bf','de8cb12d-21ee-4317-92df-23379c880453','5f05ca3a-8a5e-4853-a5b7-8c6c0dcf0e8a'}}),'92419',struct('BlockId','793c2d2a-ebd7-4dfb-b311-846f772c752c','SignalIds',{{'c2b3d6ee-be4b-4de3-95b2-89c4c1a90859','2f308f5b-558b-42d2-ab39-a19d3bc85296','12894442-8f81-49fb-bc96-47a5bf1bca4b'}}),'92905',struct('BlockId','c130785f-a926-4d18-80be-4f90a56fc66a','SignalIds',{{'ec908813-a87a-4eb7-ba88-ecd63a7b2148','535339ba-2596-48c2-be03-506c39d81c10','366d2690-c2dc-4192-9970-83448f717ac9','f371f0f8-7693-4933-881e-c0c49b24b834','286862cd-e50b-48a1-a77d-b66009e1e1b0','7598d982-5670-49cf-950a-46d2e95f4177','ceee71bf-3b4d-41ff-9237-ba63d486b492','03b4c857-d506-439f-bbeb-2927a9d31570','606bbcd9-7f06-419f-bc62-a2e7d5b97bc5','7f300e1c-8e14-476e-9a6e-132b7a79392b','df54881e-f55f-4232-b019-5e8284bdf6f5','a6f058db-147d-44be-9727-c8f0b8b2da06','7fa8db4d-7ac6-4594-8ca6-11713cd1a196','fee1639c-20e2-43ed-a8a2-8cab08ec7c97','0a709df0-af78-4e39-be07-1df5e6f1cc37','2ffc73d4-53cc-4223-903e-151a6f1176bb','2431cf26-5233-4853-956c-310646932fd2','729ed9ab-acad-4380-975d-63e616fa6b7b','d3a9f3a3-c8c1-4ea8-a243-adbe53d38ef9','05e72949-5edb-4a2a-bbd3-c4122ac77d57','d7847772-43d5-4f89-8aca-68e1f58e7bc4','0e2dd394-8887-4e3c-a652-6a7063a15d5a','ad1563f3-1fbf-4996-9483-e96b4121dfc9','4c9ad490-107d-4eca-8bd8-4fb3e5dc5d26','ac42a88a-26de-47b9-bca9-970b710b0e4a','9ca81a35-4c6c-4090-9e80-8a761f11c540','1bb2fb23-da89-42af-a582-3a530f3c8605','ecdf400c-6300-4b43-93f9-8d508bae44ca','5beee56c-6708-4b06-a5ac-337f16c18e3e','0fd0ef01-c329-4c79-a967-b8c320837d2c','c2c111cb-56ef-4355-9e8e-f09073c93074','c2f51150-e021-4ec7-9ff4-2b7c99f3ce33','848cfb17-71f4-4224-b49d-ee1edffaad9a','c4c6da3f-d096-4b8f-a8cd-fce26f2a5c87','89bdd641-03d8-49c3-b76e-aad1e5cdfea0','47dbdd96-3d6e-44ba-8764-b5359955a7d2','7fd6ed8b-282d-44ce-9b57-8d43699136fb','63de1ab7-4bb7-4e57-b981-50270329f5e6','f00c77e2-cb38-4042-8322-34274791b718','828f195f-739b-4d98-a139-038f8b78dda9','6e6f7a1f-befa-4fa6-8b36-7088daac8d48','d1eb5d09-2b30-42db-abca-b205b9df89a5','d30e2a9c-8cb1-4fe2-b6fa-254e119739a5','c50a2611-f06e-4898-b80f-d2a8b8f4b7ef','ed12cd7d-07cd-45d2-baf0-28ee0d4b5ab2','5b0e380a-93cc-4bfa-bab7-39c6bf8ae8df','5d5e6f0b-7a34-46b2-bd0c-4478dbad0934','76bfd353-8944-40b7-b49c-5700d42a22ca','8ae28102-3a9a-4452-9c8d-7f980756ca6b','78aecf0f-6640-4a27-b362-0ed6084aacfe','a4999984-1e1f-47d0-a8a7-d98d193a76ed','62717146-3e30-4b1a-a475-89d4fc6d87fe','7166517c-a807-496b-b2b0-0c8261cf298f','f291709b-5899-4f8f-b0e9-0b1bc3c6436f','0838f6e6-466d-4b57-b933-6dff588741c7','4ec091d0-9c35-467a-adde-9a2b05c5d21c','86316cb0-a76c-424f-901c-aac1475159b8','cbf9c4fe-2c9e-4d6b-a6b4-1b65a8ad655f','22fb3a2f-f9e3-47b5-ba40-49b1fc10b4ee','1dfb7ae4-a214-4136-ac0b-7079cf245438','345a56e5-e7f3-4ca4-b1e7-0f387b8ba427','3a1f1f8a-d3cf-4f76-bc9e-2a4e9279fa5f','cd2a3ed8-4a7e-41d5-bb9b-08a59a7d3e4b','f369a793-00da-413d-991a-7ce17b7db41f','18a18f5a-3fde-4178-b7a7-4e8cd440f0ea','c08b84d6-2061-4099-afc2-89a739cf1e18','7cd9bcb2-637b-4db2-8653-24bc517c69ed','5dd29306-96d9-4123-ad21-a3eaf29bf3e2','e0d9a300-19a0-4f2f-9db3-db6eda91fbf6','117583b4-d6d9-47a7-8321-f40b4524eccd','1c20b5c3-4951-45b2-8e2c-85ba7673dd2e','02b9d6f0-9bd9-4db3-a3f5-63238ae7bfdf','be4dd7e4-20aa-43a7-986e-f7667f929fd9','7494caaf-02c1-4422-a059-fe8e67d71bf6','490cddb7-96f0-4510-9afc-db0a8c3efe59','717fb977-c534-405b-834c-487b86947805','acb63aed-f138-4c6e-8d00-af2b0bbb03c4','0936a696-c36c-40f3-91df-846f868f1c7a','a9cf34e1-b783-4d8e-8eef-a56fa394d38a','f974c3ac-8c32-404b-88d7-2fd850353d3a','ab712d9f-bd18-4e64-9c93-5db8d843f7ab','eef46ec2-8c64-4ded-bc22-4c77a83428b2','499c9098-0476-4b6e-ac6e-3da4ce51fab6','96a7a772-e151-4543-b009-eed190d3e576','ba45a492-aa31-4833-8bfc-9117e61c57de','a74511be-fc26-4ca4-8c84-ec1bd451cd71','95820923-4ed2-46f9-b892-0ad0985d5707','f286fa9c-b494-4e3b-a60e-929c26b2aecd','3e0e62bf-98c2-49a0-8d63-500046b1b58a','bcafdb55-7729-4904-8359-ff440cedc889','4d105f83-f688-4ba6-8a3f-5d21d71c94d6','9eb186c8-cb59-4dff-b925-def1d565a466','7682c996-04cc-4ed4-9473-55cb75967a4a','f2685821-a8ed-45bf-b96b-32182f794528','bc60c134-412c-4d3a-bb43-1a7f4330e90f','ba3bb017-d5e1-4c43-8a70-11058f97aeee','7e15e1b8-9c5c-49b6-bb83-a58e229d268b','a88ceddc-7f82-4db3-bc17-e48d08249efe','3616d56a-cb63-41ac-bf28-51f0e7b1c317','4b29d7cc-8888-408c-a09d-3106553d5dd5','22200904-8a0e-4d9d-9ec3-ea3897d2cc15','566f40a5-b2ef-4ff0-8976-9f34c4f23ed4','1237b2a6-2799-4e7f-ae02-4614f3e09353','2c3b689a-1a1d-46e4-b759-d46a81d566a7','8eed4f8e-d4eb-48d9-9a74-9dc05842e7fd','441c57b5-523f-441c-a064-798c14426be6','869d810f-5f02-4887-a2cc-0e35a0d6e28f','5be35e7a-328f-45a9-9513-c1227225b459','5fc88af0-171e-49e2-a44e-a71acb32fc5b','a5ef5906-7844-4848-a065-698b9408b705','6e7061d7-8747-4c31-9452-ea2e35d63acf','1e735f82-2b15-4de4-b354-df60fe3c63e5','68b79d75-0583-4d65-97a2-34f06989f9ee','6c8324ef-6b41-4880-8930-eed8d254c0ac','64632b1f-dcdd-4fe5-94cc-57eb0cc9b5ba','5db55fda-8f86-4d4c-ae75-953ae856d593','c0b628b0-55b0-437c-a6af-ec6e5e98f368','741bc355-3cfd-4a6e-95a0-b4da2ba39fba','0cc9e94c-0985-4432-abca-138babe26036','5a2ca2b8-721a-41b7-b7e4-460960d9f15b','2670b056-006a-4069-ba4a-fd8995b9b55f','b07a9bbd-846b-499f-ab1e-6ff9488b5b06','c2efb6ad-b6bc-455d-80d5-ef6627b0cd88','30b3bd62-141c-4e81-9a60-af40c80f0a99','6b6a9474-b868-47ad-91b1-ebae7736aa14','496084d6-6513-4c45-b333-674bf2e18cd8','7025baf8-5fe5-4590-b72d-d86d816feb40','871de88d-98ef-40f0-b4f8-0dc1e0000a0c','f095fdb6-c1c9-46cf-9fa7-2a9700ce1846','b0e6c0bb-144f-4a95-842e-9ba7f64cd7d2','d83c4a70-f15b-402c-8b52-69b0e864f817','259f475a-962d-44d3-8b91-5e9dd09dcea4','bbc5f332-f02f-4899-a98f-b86168a0cbe4','8dfeb03b-2e7a-481c-a787-1fdf1a37c91f','9dc54510-330b-4cd8-9243-d980d190ee7d','3f18f489-46b1-4661-95a0-421e2975ac94','a7330fd8-f50f-430d-b959-09f3d9a15235','b49d1b21-6462-44a2-94e5-e81600849fd8','635a5304-d1a1-48d6-a2bc-d74dd17aba3a','9163923a-e622-4f19-a0a9-1436b7955feb','1c84b32a-25a1-4550-b1ff-064131f65061','350ac530-fdaf-4bb1-b7c9-8e535f47b8e3','8153dcaa-7e81-48ad-9b23-04e21bc6d0bf','feb7d34b-c3c6-4140-9478-c0bae6947bef','2351368c-ee03-4459-847d-a3a62a548730','5a0094ec-ddd1-4038-8922-87d7bbbf8daf','8562cf8b-2f67-4894-b2bb-7b9cf4af6caa','ea455fd0-d456-406c-87a9-a9304485aca4','608b739e-a192-42e7-8c90-e6ebcfd29f6e','3a225858-23e8-469d-b5b5-d2ac2688eaac','8a2b0f9d-32e5-4de5-bb71-70e97d623caa','b8059d39-8e4c-4894-95f9-cfeaa9c9506d','ef398a4b-09a2-4e25-8058-9b1295966fb3','d1f2e84b-7305-41dc-b011-311e002ee813','a52ffa67-49aa-4d9c-865d-61fb4d9a5296','0e85c466-9eb6-47c1-a276-95892bc6553c','d99971ea-a674-479f-9aa8-b12fdb5f8edc','97bcd7d0-e39f-40dc-b75a-14d365df892a','705d9236-60ff-42b7-9d6c-7c3a5b269b46','3710aec7-5281-4d18-b23f-3b59ce0bdb78','1b5d2176-e2e0-4e14-b081-b648e09c36c5','fc164bad-d69e-4648-9e79-81a034c0e501','1a84d032-2792-41e2-8450-76e60892769a','e7351071-8ba4-49b4-aa41-8a9ce5caa59b','547f2390-f1ce-4b5d-aa5e-28bde4c56c86','38d121fb-c965-4a02-bbde-2e1fe32236ef','19314616-3b39-4396-8f7c-99dbfc13d2e3','f4a1ebf7-8a00-47bf-9475-f932341a65b6','fc8977c3-2a0a-4f37-9ef0-236093527eca','f89eb2c7-e35b-4c6f-861a-2ce5ea019104','2db2f112-b68e-44a9-981b-98a134b0ff14','88a2b3e0-c0a9-4399-b906-1cd8a68c99db','9769dca1-5fcb-464e-9ccd-33102ad559de','a2a105e1-dd2d-476f-8470-f7c7702f3859','82b4dee0-dc46-42c1-a09f-82eb26918d2b','a0caea4e-45fd-43ef-b84c-6e5ec5b72574','b102f939-bfb3-45b1-b581-112864948e13','880587d7-5f5d-4e41-a372-6361c9666ea0','f8c2fb31-8f65-4817-aa5a-160c98555b33','a9c1676e-65a0-4699-837e-001151b9b2d3','9f421987-392f-427e-8f3d-07a4b0bb7cd6','b55a1fa6-85ee-4191-8cae-12fec46d15ff'}}),'92921',struct('BlockId','01f22f4b-6e24-4088-a5f1-2f36f2b9e2d3','SignalIds',{{'1c7f2f67-6630-4cd7-9701-ac141f1fa060','5befe1a8-1de6-4e7b-8891-44cd26086f1b','f2cc4e7d-be7b-410c-bfdf-651ddabd2b6f','ca7cfd86-91e8-48d0-bb35-e43f07627de7','bd6cd23e-0ef6-45c8-ad88-a42a21cf315f','198b6b33-8a67-4327-b291-99263e5f07ca','af908328-48c8-4bd7-a278-f0378243ef35','7201b7ee-182b-4e65-b519-5e2d619addb8','2080289b-58dd-4164-9c42-f5dfa117a957','ff43a8a3-2de7-4687-be22-369a0f2f146b','e568c5c3-2bc4-49e5-bbcc-f1dee378ae31','dfdc9c13-7a39-4e54-bb3d-a689c4611c4e','200e8c27-1d81-4410-9b7b-68163719bd09','6ffab759-023f-4394-bb47-280b66ffe6b3','76a49c8f-edc1-45e2-92a2-ab0d2f5c4e91','ac2073b2-bf44-4b11-a393-ce15245e2cfb','3d976923-b171-4f4f-8076-285e1bde1139','baacb540-6ff6-45d8-86a4-cdc7dca80cc6','649ced62-c471-4600-8cd1-09c0eb4711cc','a0358286-2848-4d87-b0b8-a452d46221a3','d803190c-f7d2-4619-98d1-4c4b734baac9','da135805-cfa1-4dbf-a174-45767d6826ea','c611273c-765d-4cae-9a59-66522cbb8f94','32bef2d1-e4ac-409a-be5c-e1c82092833f','4794b83b-926e-4eed-8f32-dda74d7bf2be','e3a799b8-941d-456c-ac83-3386fee11fc9','ec3a0644-282d-4554-af68-83c7b408cec9','f21e69d8-af9b-47cc-b57b-da86072e24ee','7d2f16bd-ed5b-4114-b605-0294ce439d80','cd66ad97-a19e-4182-947c-8bcf9e691bba','e722b9c1-e628-41b4-bad4-7d04f32338ed','4f01fabf-ff54-4f11-a3ef-d08fbfcadf3e','56c3e53e-96bd-423e-8d28-cbc71941af08','021ae82c-3d62-4cb3-9e47-c34e9e3d0ee7','90119441-15eb-476a-a3f9-98d0cf770601','b34b77aa-2a3d-4a61-bdc1-5546a0039aec','fcc0a909-f3b3-4d49-a3f0-262611af776a','c4b53111-e775-4e8a-a4ca-3136addd0276','87e1c377-552b-41f6-8293-f718c1dbcf50','f011b660-9889-48c6-8da7-8d9c66c6ad30','4cae1440-06b8-456f-bbdb-de69bc1dbeb5','ebb4632a-fa9c-4516-943c-02ae56da63c1'}}),'94738',struct('BlockId','bcf3b81c-74dd-45df-83eb-246bf1986e5b','SignalIds',{{'df4c9189-aad0-47af-adf9-452f98c57b31','590484b6-080e-4efb-ac1c-229f01eeeca2','6c31bfa5-0aeb-4eac-8963-270cccc0c2d7','5d56885d-f8a4-4ee4-b27f-0c2d3ee21fbc','5ee8659b-4f86-4877-ad6b-d7985f9a954b','5766d64e-9371-4170-8911-2778a90268a1','ca1e598c-d3c3-421e-9ae7-e7185f2a09d3','18fd676d-98a4-45b4-b1d7-9d0dddbc5e6f','5fed29b2-e1d1-413a-a8ac-edff34823113','279023a8-7daa-4d97-b9e1-4a91dad2ee5e','cf1bf694-ae18-42fa-a463-b9dc6cafc69e','32f22328-8598-4806-87e2-5e23a0c26b38','d9c23c5e-7a50-46d5-a10e-63ab1b9fc3b5','cf79ee48-71f6-4fd0-8aef-9c9bc30a4e49','611bb3a5-99ac-46c3-8b8b-53585c164246','d4d01821-99a2-4800-9374-6d86adaee4f2','773a5d70-a4f2-4240-9854-c19ab4783338','36678538-4ce8-44f9-9a3f-03d3e9efb7d3','ff0c1d1c-6e4d-4843-b338-e274e9a45ea7','fccb9dd1-5cda-4fe6-98ad-c7d4fc6f6931','30094c6d-d28b-4ad1-b945-e3ec2bbb07e8','fd218d85-a724-4108-b9aa-9a62089b89af','31fb8c44-bb36-419b-9e97-03acaff2a29c','a78c2e56-f9ea-44d1-b5a5-eb44b54675bd','82bf71ac-a176-45b6-9db1-c74f24b49a0b','44157694-ff9e-47f3-8066-6bd1e0cc2fce','893b8782-7964-4c73-81ba-5eb32773f42d','d274718c-9e26-4b13-ae78-5a9d797416c4','f6cb9ef7-9823-4ce2-9c69-15ccc098452a','0a99d19b-e178-42ce-b1dd-cb3f737a3d84','0d302e1f-b775-45d3-b6c8-d5c622d2f19c','c39d27b2-dc5a-4618-9837-71f8924ef39a','762f9018-3929-47c8-99b4-a7a3b2c20982'}}),'94769',struct('BlockId','ab122073-fe81-4e3c-a510-f985427cc27c','SignalIds',{{'5ef45bc3-f82f-4f11-8293-37f21f3ed968','ada81622-287d-4c74-9c00-6556f221b335','5e588d7d-6005-4734-bf0e-fe75e130e906','479383e5-dd07-4660-a182-a5d6f9c4f86f','0dc36b3e-fc07-4ded-b905-8f085d96a787','7352a0aa-a73f-4a8b-a120-1075c01938c5','b3f3e0a1-baf8-4c8e-a86c-29d225bc0e37','50d9c351-1646-431c-8cc1-f926b0084f1a','65bc14d4-7425-4c94-8508-c951edafa4db','11fd3803-ebfc-4b14-a576-ba1381606d34','3f23f25c-0dc5-4753-a10d-882186805523'}}),'95726',struct('BlockId','ef0b5d28-b6d4-4eaf-949d-d6dedf719559','SignalIds',{{'ee15b610-82c6-43bf-9a8c-0e7a9659ccea','3b41ead2-8f03-45d4-b3a2-152baba76f1c','04424910-0e7e-4b8a-bfb7-18efea10e449','d3e92efb-eafc-4308-a397-493fc39ce811','878e6af1-c668-4ab0-8e4c-5c6032b55278'}}),'95727',struct('BlockId','b2b56e4c-9e5c-48f2-8bbe-9899bbf5491a','SignalIds',{{'4e2474d8-d594-488d-9a95-ac26de9b628b'}}),'97162',struct('BlockId','609081e0-941c-41af-a124-0ef5d7529c4e','SignalIds',{{'7a0f8b5e-91b5-4be5-aa3e-8b6fa3ad27d1','46832e0a-dcde-4f52-aad9-ee2d5b2f815f','bfa458bb-0f77-4e22-9fd1-ceaff99b329a','ac728005-1b3c-4171-959f-ae8eff693e6b','008a89bc-e3d6-404d-8ad8-0ede00b346c6','21c71be8-3a66-4a2c-95b9-571df8448d55','201d8bfd-af86-4d0a-bcf2-2be355973df6','17b8c076-2f41-4633-b3f4-ebc4292cdb2d','ab00a850-8ce7-4b74-9f89-de7c76bd9fd2','240f9350-204b-43d3-8912-096b8d4fb3f9','cb628a66-37e2-44dc-ae8d-af5a0f7c0f4a','6af2e867-4ffc-447d-ba29-ba8626120048','9fcbe341-bbba-4ceb-b6e8-1ea49d1f1c20','a24cecca-e5e9-47ca-8406-22f227da4bb4','664c1055-c028-4f6c-a847-16dc729d939b','94775a18-8b75-4854-8d5a-a4dd0e581b4a','232f361b-601e-4443-b8a3-d4bc6ac96435','1fe87f67-5efa-4bdd-9d59-3c81b1c88557','81f862d0-8470-4c56-9e69-bc32aa30d43b','e1a68ded-277f-4555-a456-1524c13163e5','eab70a40-031e-4639-a10d-e5d41cb3f774','f526a80f-9956-4640-ab3a-89d2045f0162','edbb942e-05fc-4847-8de1-9a53f76b57c3','fa5191a1-3a1e-4763-8ee5-164c10c89699','50910d49-eab0-43e8-a422-548b52d3ac7c','0663fc9f-f5a9-4bfb-ae5e-87e83d32350b','eee09491-0338-41a4-874f-f2316d53c699','6f8a9a16-516f-452f-b2c6-592de3d56c59','d4fab639-aa70-4ab6-9a17-13486f62d987','8d916867-5d55-43ca-9700-dd7feeb9bc6e','eeb9a4a4-84f7-47c1-9ce7-0ef2f39b74ee','730cd9b7-4ed1-47c8-abb4-845d6e05153b','3a8d6f03-c7e0-4aec-b7ea-561ca6594a58','25840a63-a918-49a5-a812-8a1a8028e971','aef27282-f49b-416e-827e-cdd345ba9667','24938d64-a0e0-4af1-a018-252efc3ebd59','e37b8316-1f35-4643-89ab-21172ceb4edf','b22000d8-6743-4f74-a74f-a3205d460f56','071f6833-b20c-4d46-b3e4-10e823412cbb','ec3e142e-8960-4688-a09d-a55ea4e32adc','ad9531d8-6532-493d-beff-fe127dba79c1','d835263a-ecfa-4975-9fdb-449f341a58cb','eef83801-769d-4b17-8c33-06ecd7e9531f','5d0189f2-7d3e-4f08-8fe0-161cf62f662c','d2f707ad-9b49-432d-acdc-bfb37fb60912','1a39fb43-09e9-4f77-8799-5ac95783bd7a','c7276a0a-abe3-464f-bf0f-2f48a797c1e4','bd5870c5-724f-4d37-8fd7-060d6b5b46de','d639d805-c587-4e89-b332-581ad6e75f23','6efa384c-85a9-4595-b0be-cf78e9440493','53d8dcd7-0a8b-41a1-a4d7-7828db180377','9e7caebc-7806-4f8f-b588-3fafd79f3b79','2e9b888e-502d-4f3f-9192-523b6326006c','12683d1d-dbf1-47f0-883d-2f89e9585a50','0247e252-86ee-4c9b-924e-349beb4cec5d','dc694a7e-2623-4887-bd95-05da09f2976d','ebdd29c2-8c6b-4b33-8057-4a6975ea33fe','858e3f46-3ea8-485c-b4ce-1dbd84f5f4b5','bd26857f-1a73-40c8-81ea-009552807393','a67ed66b-0df4-4077-bdec-79f7b0742a37','41ba233e-5517-4492-8c6f-88d14ae87849','e89fef81-5e13-4cdd-8565-e3a4bc554c6a','79d59ed1-5a59-4091-a0a9-961027512cb9','3157c6c1-20b0-4cae-80e5-07c8fe13cb5a','96edf60c-decf-4636-b100-d32d9156fdc0','0186c05c-0b8a-45e7-acad-09290f940f36','8d0919bc-d469-4ad3-8876-2215fa1e3c58','94796f50-aca0-481f-b09f-bcd3b61dacf6','0211f4a6-eb10-4ff2-9ded-efe2f54bbcba','3fc8fd11-180d-4279-a4d1-d315f519dde3','95a29aa1-566b-46d4-92af-bb59b0582c30','74c5ffe1-f404-42ea-bd01-db28b37aef92','7582e1a1-8611-4d3c-b4a0-d1ba90126ba8','a38867d5-0379-4628-b738-91d324b276cb','1aeab194-b8fa-40b5-9dd6-7e24b15055ed','e65d4b7f-5403-4cfc-8754-8de4db2dfc3b','ceafec07-8674-4c62-89be-392175838a4f','571a7066-71e3-419d-b801-ed3605b6a94d','a339d5bc-4bac-4202-9add-1e8b4b128418','38834dd4-1316-404a-b5fb-2b6d10676a60','28b836e1-ae50-43fc-84d6-d9ce7b6871d9','7e48a4f9-6a73-4625-9ca2-29b40c8ff1d9','a2bc4953-5b0e-4e1f-b774-6d10007aa0a6','f286eacb-0890-4462-b3f9-5db0fafdecf3','86954f5f-41ea-4f72-bccd-7539044883f7','da475526-0c4c-47fd-9fc8-9468cf6b7138','eaf5dcf1-085a-4450-95d8-e0e1b31b251b','8df4d6d9-a5f5-4230-9551-006ec052d287','a6905aa2-b44b-4297-9a6d-b056c9f0f561','7c2775f6-bb4c-43c9-a1c8-611712bdfe50','f8aac724-2f6b-4507-96c6-fe2b499ca7af','c6c5d193-f81c-4525-a928-e534762a4996','1b3b3208-9784-425a-91f4-316eb01c5c0e','120ab8db-7f87-4a6d-80f3-9796dc49379f','6d4e0623-c660-4980-bc46-d841b5f15fbd','196c7c87-e6e8-439d-9c9e-2d0be2a1badc','914fd7ff-ce5e-454f-a0dc-6be5016f04e5','8fef58bc-aa80-45b7-99ac-679676dedd7e','dc22e312-d229-40ff-8255-43c4024e57f2','ea3a9df2-9771-44f4-bd80-87ab18d08c8f','d45e7130-805a-4cda-94b6-fcfd560accf8','332ff65e-4f46-4811-9c0c-aa49297458b8'}}),'97187',struct('BlockId','28a1268d-6eb1-4b71-b208-78f973de8d60','SignalIds',{{'585913a2-9f2a-482f-a871-6411ccfb653d'}}),'97198',struct('BlockId','d5a98707-e9c4-4286-94a2-1770c80d7f4f','SignalIds',{{'c855aa43-135d-4843-9f79-db840653e8fd','54417ce3-4c9d-44b2-a33a-25590b836b81','47cdef3c-44d5-42c9-abab-8063e32dbde2','c6425e0d-8cb7-4b97-9fbe-624d35a3e47c','77d2dc99-15fb-4ca0-8459-b10db5f54984','b06d46da-0afe-4348-9620-4a48ae4589bd','99f6435f-1975-4fbd-bd5f-98da826c52d2','e20ae6f0-ed78-4f04-81af-c59b4fe103ab','bb3ddaaf-07fc-4bde-931b-8b2831ae140f','369e9b5a-187f-4111-aa6d-64fcaeeff6b6','0600b854-4b29-4c2c-b5c2-771f8ef656ef','3d8d12ec-590a-4d9a-88fa-80749b59276c','a3bfa13b-5373-4658-bc35-8787c30741b4','b6e39718-75c0-406a-a8f9-b4ed2f932d63','3ae9b18c-9a42-4f93-bd17-c5884e555cba','4407ef51-ef66-4e3f-8e23-bf2f84b36441','80162738-9f36-41d3-bbbc-cd6f71812cfb','145ed585-4889-4f43-a872-6ebb3f7d528f','14ea400c-c0bd-4096-a660-ed8b908b94a1','e52b016b-0789-4cda-8e41-4c5419829fcc','d084e8ea-b9fd-47a7-a81b-404462515d73','14127863-cd8a-4aa2-ae63-f72ff16a2976','4d6dd348-42d5-4e2f-9857-af5495f942fc','9e1ffb98-cd10-47c7-bfa0-c7f82980d00f','ee3cfac1-8666-4d88-af2f-dae314b9dab0','32809660-4ebf-40a4-8fac-00ba1a8694bf','9df86f16-1321-405e-9e8f-6b65c0a77fa6','bd514d21-f259-4ce2-a044-75cb8241019b','4846c61f-afc7-4cd4-9014-9664af955811','386dabd0-67fa-4157-877a-5d180a615039','49f7453b-7d25-4dfc-a6e3-96b47f9572de','b88020d8-7bff-4d0e-bdbf-e55a3db9d2bf','f1b13c7c-ecc6-411d-82d9-5440c55df978','13a9fac6-3b2e-4e20-bb2d-49a8badf1a80','26f9ad9c-eaa6-4a90-a5c3-39f447a9ac78','0af830f9-f5e6-454f-91de-cd60639fa1e7','0560ab11-f83f-45da-9f12-4a6919fd4ced','29d2492e-438e-48be-9926-d533d6feb313','872e73e5-2920-470b-9957-414be0968712','e5f43741-853f-41ce-8e42-68a48f704f7a','43f3f7f5-28a7-4c90-a4f2-0b63d3a25f7d','a968688d-5a25-4c23-a524-134b79f7ae05','675b099e-8b6a-41f9-b872-a4bbd499150b','2ef6222d-d808-4404-8286-93450e58a407','6d426830-ae0e-4b9d-8b8e-c7a48734a28b','9d5335f9-6bfb-4110-bc63-fbe87897593b','b9f0f5a5-b551-4e47-927a-8ede67aa92d5','9afcb1de-463d-4956-bd81-daaadeee848f','22d4c151-a8b7-4096-be9d-b0fdf8528350','edfca5ed-cefb-4e7a-b682-09011c6dd0a2','27e13cb0-125d-429b-bbfa-79cf555714a8','b14b42fc-9505-403b-91f6-3fc60f9419f1','f11f7922-4891-4d2c-b4eb-aab8199e3756','1a5d8126-688f-4f87-92ea-4dfc2f81fe73','07a9e82a-eb3f-4b00-8031-1d46832aaf29','fda4505e-cb50-48ca-bcfe-4ac1460b16e2','3b2e4117-90d3-4408-94cc-bf1633040885','b0df4232-7da3-42ab-9f51-717797e8d978','89c96393-e15a-4f8c-a0bb-5addec976af0','ce89c7d6-af94-4858-9886-ba85618ff3d0','97b14e89-7e16-45b0-abcf-7b63079a139d','2959c2fd-b9c4-43c8-ae3c-0bf737823b3d','7b7f07f8-d0af-4756-8660-6fcbc2323be3','44f08197-78c1-4d08-b16b-972ccb00d32c','47ccc443-dbc0-4163-b94e-3023e1cc90f1','fee7ad07-4aad-4075-899a-d709b7f73b9f','b80ed905-e196-4089-9d38-a63c4fc3e0ff','eb35c15b-9175-47d7-a1f2-71b557a9f887','6ee26301-5de0-4a4c-876e-bac75a633ad9','e386771c-ac00-4ed2-a2fd-067c02672470','37b5cf25-dfb5-4e8f-8246-fceff19a7fd3','2b936f37-24dc-43ac-84d4-c56aa3fe720e','3931ff07-50bc-4616-823f-daba0e6bf238','3ed67b90-0b05-4a41-804c-27b0d840a85c','c1b8f6b0-29a9-4807-9733-a3d0e1039b03','067383c7-cf9d-42c8-a878-9e46b76d93a9','71f564a2-ab04-47b7-8890-1fd2a41ba090','8314a54e-ae40-44d8-bd1e-e3d36f768aa9','ba08720f-0ff3-454a-a0d8-77c8e3624210','65821741-3b91-4356-ae05-456002bb6637','013b88d3-b79b-4d63-a4ba-78498664be62','11e467c6-4f8f-40a1-bb47-6f5534593064','86b552e3-fb0d-42e3-ada8-6fb503052d11','306eb17a-03b2-4afe-8c47-fa019acc3e5b','5f9aacc0-8a99-400c-8122-8554c024806a','1c4ec95f-4377-4e8d-81c8-17e0409e5374','d5f1f4b0-a4ec-4d78-9136-f7381469164d','1932bda8-ec34-4aeb-8f11-f5cdfad08262','ce1a3840-3719-44c6-a444-2d6cf192911e','c028750a-bb52-4abf-932d-7b5a6a5342d9','87183d5b-ae04-4daf-85e4-c88dec1a53fd','8009f076-f77f-41fe-9ff8-e2e1c0c42177','5940b7e9-f37d-4acc-ac5a-f3f10831f659','1561e29a-0bae-47e8-bccd-698a30165295','74a6ff88-a32f-4536-99a7-5c33638ce392','afdefe1a-e3a3-42d4-8967-c18a8b333b14','241b2513-728f-477b-8232-42d66631417b','28b79b5a-055a-4112-bd05-df066b9a7adf','fc21657c-150a-4547-8e02-1f2f56db70b4','9574e010-78dd-4311-a59e-625492259326','b264e420-53d2-42f7-bc0a-3d486e1f3dcf','b1a0c23e-c8e3-4cf7-9b86-eac31ff31471'}}),'97223',struct('BlockId','2bb0817e-a54b-4064-8246-157ce30e8a45','SignalIds',{{'7c35180c-1def-4620-8cfc-ba0748efa5e5'}}),'97304',struct('BlockId','4118e63b-9826-405a-808d-6a2815e4502d','SignalIds',{{'01b3e1a7-f378-401f-8832-c17bbb23d801','8bb1a5ae-2220-4e72-911e-1bf42e58e4cb','dc537a66-3ee7-4b74-a769-466a6749f5f3','cc345bca-7163-4f98-8c36-d8b285b2316f','72bbf11b-86b8-413d-a3c6-b15ad8f593fa','09d8c20e-ec8b-4845-87b9-7498aee8976b','6f95cbe8-f55d-4f50-9a94-a1486b31b339','e42558b7-a07a-4146-9aaf-d538d4bcc547','a567dfdb-8fcf-4ff9-a1d2-e4b8ea8e87b0','a4a04237-9ad9-472b-9cc0-cba6eccda89e','d21b2fec-157e-4546-99aa-20a49f5b2123','cf30603d-a017-4758-b4ef-acc10542d365','f97d1c5c-89fc-42d1-b443-04b1f4566020','e5ae5f93-2521-445d-a42f-5357582259bf','1b59a933-7082-4e42-b5fb-636e4d03095e','2f90ca23-1adb-46b2-86d7-31ad12da6482','0f36c745-20f7-4ef9-9082-da06e169bfa1','061d2dc9-9131-4b99-b48a-9b0ff8d8b97c','28be56c8-312f-4e5d-b18e-1edfd44a6e2d','0e79623d-4bcf-4cbc-8070-38f639d67d18','908c7efd-3bd6-4f85-a3b6-9d52056e9c78','1cca5fa1-9e04-4d62-9101-d6ee7080ce3e','a775926e-0f86-4205-af19-7b70071a253d','19793d7c-79d9-44b8-b460-0f82d260e67f','9ca958bc-1b2b-4afc-b1ae-7d8be721e757','93e3fff1-70a8-4a0d-9417-b9de293bd010','ba446519-3a3b-49ac-89b8-b12cdaca3106','b73d54a4-a414-4181-944e-1eb485d8283c','89d5975a-ae08-413c-887f-694367b6d4b7','3175ec4d-6a41-4088-a19c-d2366275cf89','03dd4b3b-b690-4de4-8e85-f63146e35258','60627bdd-944c-4e63-8d05-4ea0006561b9','7cfda0de-925d-402d-9482-3f6fb5c606f2','240cbb01-d769-4a55-9c48-191c9f95868d','6832e2d2-1db0-4b5b-acef-28d647aab0f2','677c103b-6c9f-4bdb-bfc7-6fa9b6622754','cae61037-28de-4d53-8c0c-8a4e07abc496','1e5e87e4-d961-4212-b768-b5a8cdee5839','d5531e03-5688-4968-aa6f-7cc3599e3350','92e24c3d-ceb9-4877-95bb-ac81a5f8d155','6a1b7d30-ea42-4d8f-b0ec-1e21fc93c1cc','4559e5c9-5dc5-4cfe-b9b4-35e2b3daf863','c80a97dd-3775-4c55-94e6-856feacce23c','1f4b3783-ec57-48d5-bda0-a9f90bd3245e','9163066f-f49a-42a1-9a3d-15ea6dfa20f7','b291e216-46de-48e3-bdce-9d5f83f81ce6','7d72d178-26c6-464b-baa5-cdcc786b292a','b93ddeeb-1b31-48e9-b7ef-934d2a9e5c49','ab219c3c-0350-4a60-97ea-db06c4fee33e','6e3b383b-48b4-49c5-8c97-d9f877d2d3cc','7b66c355-0d89-468d-896b-3bb056f5e6b0','3b02ee0a-f6e7-4055-8a74-f81765a62fa6','98edbac0-0bc0-4275-b67e-d83d083685de','f12b0a52-09d5-4ab5-95d4-376bf9cdb91f','58e7d122-3c14-4ec9-be76-5a19bed4fc74','545ced7a-c299-4d81-a823-688beb87c278','8eb9c465-bca1-4103-bc99-d8a256cc79de','13a7d792-0e73-4cb9-8b76-7c831f116066','505c70cf-0ebc-4438-af82-c82737fb82b1','36cd3976-7cae-46c2-bc66-0783780c46f4','44ad4cb4-78fc-4870-a22a-c5737ca7506e','0f308031-0ae5-47ed-a451-2b0a8e74e6f2','69f4f3f7-67b9-42dc-bc25-a8b39ba3090d','080e6084-e7a7-4dd4-8b1c-1c43e9dcd6ba','74a9494f-9873-4c2c-ae76-8a0f74db06d3','ccfa1334-ed0a-46c5-b27b-0d24b3fe104c','02647cfd-7651-4591-82c0-c306a45d9954','bf5909b8-e47a-488a-97ac-8a8bb4162d68','1b52b0ef-86a9-4dcb-8cfe-32aac3b81ff3','3598f962-26f7-411e-8435-40818213f22b','1e0211c5-e0e3-470b-b0ee-33e8bcc4d108','5c746092-0c30-4e69-b43c-c92dfadd0b45','d778509b-398e-4732-8971-0ff5cebf9cf4','04576cc4-8882-4415-afa3-aeedc508a3be','c024dd67-34b1-45e3-a631-5b7bbf918376','11631a09-793b-4867-be22-79d9d65612c5','a3357929-da2a-43be-aedf-f6305debcea6','de752852-aa1c-48f2-8ef2-374d2db6bf7f','b12e6e17-85ea-4152-b69d-d16c6eb749a6','374358cb-0fa7-4c8e-92e9-037c0bb44a3c','1804bd15-cbb0-4ab3-beb3-6ef8ee465187','91472f63-d464-4e24-b37e-63823e391a72','373b3a93-b019-47b7-baeb-06c0a5a55f6c','814253fb-3bd6-4d1a-a9a5-a3f852134056','3b484bf5-91e1-4a0d-a7fa-cc4fb327c5c5','ab27b948-cf6e-4c05-947d-dfb2c65438d1','2f1b953e-1e5e-4065-9a7d-c6a7bad72005','a9f5e343-41f1-47a8-9445-7de5b8319862','0b7abe1e-ae09-4c9b-b38f-26afcca63e63','120ec359-a99a-45a5-8978-ec6ad16a0a24','a1386bd1-b3cd-4f88-82fa-66a9c6dc047d','27ff8947-825f-4a8d-b1c9-e78d91e1fc65','e484b846-ac39-427a-9333-a5dd0679e88a','a023f569-8a9b-422d-8e35-98d8b20c49a0','c6fde034-a3b0-4ecb-bb08-4786cdc61482','1ff15978-77f0-4230-8db7-739deffe4e18','2dc576c2-15f5-4b47-9974-0fc4caecf4ae','3c460159-3a51-4504-a157-b91f565eb795','5d8de635-6c66-4c6f-a0e5-69443bd37ffc','9f232409-b5b7-42be-b408-d2f2a0fdf988','0d56aaad-3931-43d6-9944-cd7d8d94e774','7ae3225f-bf53-445a-8835-56fb9d6975de'}}),'97309',struct('BlockId','c5b8f01c-70df-4224-b497-d544796a9d10','SignalIds',{{'42317a15-fedb-4030-9b34-a5b724ca26dd'}}),'97340',struct('BlockId','8b0a5312-a67c-48a9-b34f-1d6be82c8843','SignalIds',{{'f4db5faf-fb61-4c6f-b640-80cc192d1c8e','0a8a547f-22d8-4376-a9b2-5714083fb1f0','1208775c-8773-472a-bbc7-698634299448','ca05a6e5-cf91-4f1d-bc4d-28b1eef3c49d','d8eea1a8-aa7a-4d6b-8051-6bd9b610858c','5c7a2e4f-ace6-4026-a188-f979e1be3eec','bdfdada9-9c4c-477f-911c-c65d9e1ff339','2a208145-772f-47ee-9a7b-1aac75928245','0241cae5-c55a-4a65-bb99-da8f2c93baa4','4eb98ae0-8f8d-460c-87e0-ed84f1337715','a415dc3f-993e-4c04-8f62-408ce761464b','9ea75a97-370b-4a3b-9631-8371a94bc6e1','bab598bf-ac29-4c30-89d8-a221a5aa8c31','1aa88398-2c2d-4566-91b1-886bf2739ca2','435cceb2-096f-461a-97e2-2803eba8e13b','bfe550e3-05f8-43e0-92e9-29a659165fe0','575066b2-5f9d-4f7a-aafe-06d054514401','1708d4a7-b108-4092-a880-4a9233a5db3e','73bfa96d-f7ac-49ea-ae1e-07195bde5abb','74affeca-f459-4b5f-86d0-0c77c6a80cbb','bc634706-744e-481b-b24b-00ee508eb29b','740ee232-137b-42f6-a63b-d6fc7bc48afd','12569f31-0a11-4715-ae9a-329e667c8980','e6c015f0-2974-4f95-a10c-da91412374fd','4387b9aa-8d23-4a34-abe7-732fb690422b','053a1b06-d267-4261-ab75-6cddd42f835a','7ec7c7a3-3230-4240-8e12-f8259b3e50f5','4e427f28-e16d-409f-8c34-1cf947def933','4334d358-33b7-41ad-b6c7-bbbe6a15cd96','641298f3-8099-4649-a67d-48c86f0109c3','fece37c9-e9c1-41bc-9561-ca5167e3760b','c3eb5f33-0244-41d6-b000-ef71fdcec568','0423900d-d6a2-47b1-a914-20055e321f8b','2a8324e7-3ea8-48b0-92e5-d055fbeb7eab','6642d8fc-9171-4ea0-b94c-c96c126fc14d','3576bc2a-e5e0-49ad-81cc-7ebab95dd16d','d2b19811-e4b0-41bb-8d49-39b3e6b99fb0','915508e0-5c5d-44f1-9d3d-642b8c880c17','d8b08ebe-0925-4d0b-87db-03c30dda66b9','f4818373-bf5d-4163-89c7-b21ae55be742','96242654-5563-4c8e-b566-d07fbfac1306','23f357d1-3449-47e0-94f4-b286c13fb786','1ba80edb-a9cb-474d-a9e6-e513b0603c58','310de9ef-30f4-4123-ad2c-6c3e2bb8cdb8','20562b24-0576-4fc7-b017-69f3f3ccc63b','798f6ac9-f091-40c9-989f-56db13ad6a47','6ec9516c-85ea-45e9-8ab4-0093f3a91e2f','9df7552a-31cf-485e-921b-df523f724704','ec138bc5-e3eb-4cf4-87d2-e7579a9f6251','af8cb284-e6c3-47ca-b8b1-40c443f57341','64a642ba-e69e-4880-922c-edf34f504555','171efce3-6c24-4374-80ff-f06938082a4f','ceb2b419-1ef8-41f7-bb11-9d18df5d57c7','b8697e03-5a59-4bf1-aad7-541e0428d259','362a533c-6a8a-4b17-bc3f-ff9cfc142db3','82f7ee3c-0c78-4ac5-9a90-504c6e1c5f61','a3088f2d-b3a0-45c0-8664-b7c71dc4cd0b','a5de082b-ecad-4b6b-ad31-be924d507c77','7598d421-a0de-4f2f-ae81-e6ad1d58678f','24ec6dbf-6a7a-43fe-bde7-da8e87280e0f','46d535a0-a696-47b9-b3fb-1c245866e275','66d80951-c89d-4662-a7c8-904a0ad9de4f','74d4644c-6531-47cd-8e38-a372987bc87e','9b85a97d-7784-4d81-93b2-842cfc9a913f','1ab7e146-7e4b-4998-b71a-3d7a9edc6f17','f0c364af-fa8a-4c8d-8510-3d1ad58b3dee','3edcede7-5fb6-40ae-bb74-45748a2f8b04','ebbfa0b3-96d6-436f-83eb-7df4fa5f1753','31c0be34-4583-4914-bbf5-fd00b1eff51f','37146b77-3cf6-41e0-9f22-ebc5150e8b55','3c486663-aff8-471a-816b-32755038f8f1','27b815e5-a0ce-4c30-bd2b-26d85581817d','f7166b7a-6973-4b39-a16b-b8fbe3fe9cc1','feea72b2-2773-43a7-99af-916ac0b76199','eccd43b9-5fe5-4f61-9037-958e696fe794','89d86823-deea-4f9f-8fa8-aeb5a954e9e2','c116d586-a9df-4d63-a2b5-7e5c433d34c9','867b7238-5ae5-4938-a9cd-68a740cc4e21','b9c6a7e6-8024-4711-afbe-1f7024b054c4','08ff8eb0-eef2-4cd6-ad6e-24cfede8dc88','0c7c8510-5563-4676-8959-769a06cacb80','3ed829cf-810e-453b-9dcb-e522b81344b9','4759b5fd-55fa-4029-8b2b-8ea57498efe7','3a2cf3e9-867c-4245-aa08-7da53a1cddf0','05aae4f7-de30-4e26-96a9-a4f1229cc9ba','498ef53f-2fe5-4b37-8cce-a347fe2f7864','193065b8-1e38-4271-8a34-6162173ab439','e87822bd-65e9-475a-aab3-039336777ec6','a8177ff6-52df-4029-aaff-fb67f98b7c63','3f2bc1d0-9331-4d92-9e4d-7c4cdc2c3d27','22121808-fc8f-4e33-a24d-5cc22ca05efa','4faa7336-d281-484e-ae56-18def0883cac','e204e675-27e4-448f-99f0-12aa4c9f43d1','ac3856d2-afc3-4a11-b9ee-a103cba9d318','54bf5ada-91b3-4715-b3d7-7280f1698d9e','f868dc83-b00a-4e3b-ac80-5cbf1894bbd4','8bb4a648-1d86-4380-970a-d73ab9d8a0e2','bff3fa35-78e8-46f9-af03-f4eb9ffe08c5','88948313-4a10-4073-847e-eeca1014f4fd','07021bee-bc6c-4722-8770-202430afa4ff','29edcd57-f9a1-48b4-a543-d113eaf6794e','9f9f5584-5b25-413c-aaa9-bdc9a63feda1'}}),'97345',struct('BlockId','e0f8d838-16b6-419d-bd34-87d4e2e4bbee','SignalIds',{{'bd79ff19-7d83-4483-bee1-28b1bd8e11f7'}})}  OrderedModelArguments=off  Creator=GW00133806  LastModifiedBy=GW00216231
settings OptimizationCC: BlockReduction=off  ConditionallyExecuteInputs=off  DefaultParameterBehavior=Inlined  OptimizeBlockIOStorage=off  BufferReuse=off  EnhancedBackFolding=on  OptimizeBlockOrder=speed  DifferentSizesBufferReuse=on
settings DebuggingCC: UnderspecifiedInitializationDetection=Classic  MergeDetectMultiDrivingBlocksExec=none  TasksWithSamePriorityMsg=none  ParameterTunabilityLossMsg=error
settings HardwareCC: ProdBitPerPointer=32  ProdBitPerSizeT=32  ProdBitPerPtrDiffT=32  ProdLargestAtomicInteger=Integer  ProdWordSize=32  ProdLongLongMode=on  ProdHWDeviceType=Custom Processor->Custom
settings ModelReferenceCC: EnableParallelModelReferenceBuilds=on  ParallelModelReferenceMATLABWorkerInit=Copy Base Workspace  ModelReferenceNumInstancesAllowed=Single  PropagateSignalLabelsOutOfModel=off
settings SFSimCC: SimParseCustomCode=off  MATLABDynamicMemAlloc=off
settings SFSimCC: SimUserIncludeDirs=|
  | .\McuEQ4Parse\src
  | .\RoadFusion_L3\src
settings RTWCC: Description=dSPACE Run-Time Target (for VEOS on Windows and ConfigurationDesk)  SystemTargetFile=dsrt.tlc  GenCodeOnly=on  MakeCommand=make_dsrt  TemplateMakefile=dsrt_default_tmf  RTWVerbose=off
settings RTWCC: CustomInclude=|
  | .\McuEQ4Parse\src
  | .\RoadFusion_L3\src
settings CodeAppCC: ForceParamTrailComments=on  MaxIdLength=128  OperatorAnnotations=on
settings STFCustomTargetCC: TargetLangStandard=C99 (ISO)  ParMdlRefBuildCompliant=on  ConcurrentExecutionCompliant=off  CPPClassGenCompliant=off  GRTInterface=off  SystemTargetFile=dsrt.tlc
settings GRTTargetCC: CompOptLevelCompliant=off  ConcurrentExecutionCompliant=off  CombineOutputUpdateFcns=off  MatFileLogging=off  CPPClassGenCompliant=off  UseToolchainInfoCompliant=off  GenerateASAP2=on

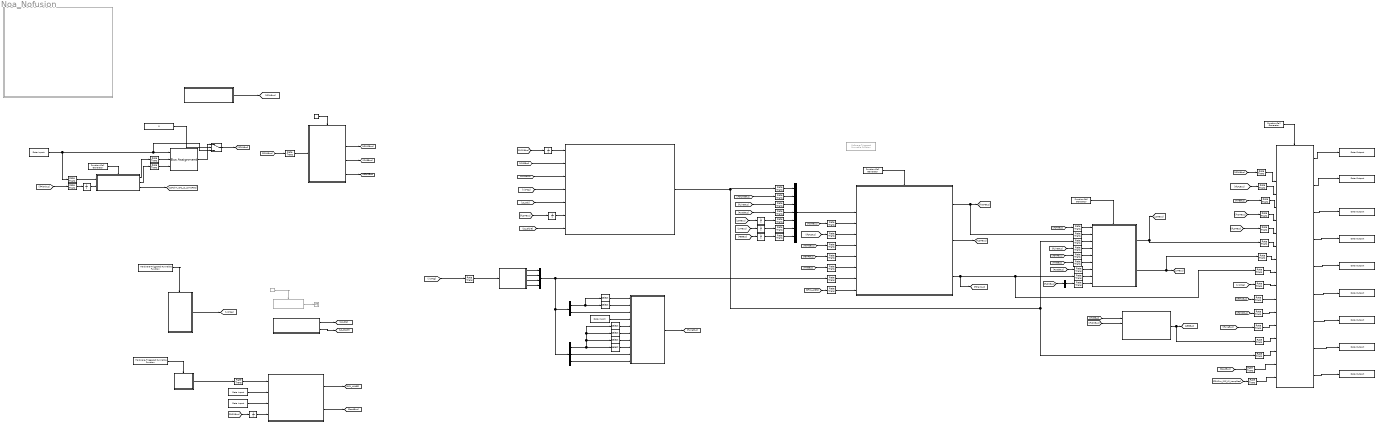
== system Noa_Nofusion ==
  note: UDPReceive
  ACC_FD1 : dsmpblib/Data Outport  Priority=-10000
      settings: SourceProductName=dSPACE Model Interface Blockset
  ACC_FD2 : dsmpblib/Data Outport  Priority=-10000
      settings: SourceProductName=dSPACE Model Interface Blockset
  ACC_FD4 : dsmpblib/Data Outport  Priority=-10000
      settings: SourceProductName=dSPACE Model Interface Blockset
  Bus Assignment : BusAssignment  AssignedSignals=CSA_NODE.CSA1_MSG.LTurnLmpSwtSts,CSA_NODE.CSA1_MSG.RTurnLmpSwtSts
  Bus Creator : BusCreator  Inputs=7
  Bus Creator1 : BusCreator  Inputs=4
  Bus Selector : BusSelector  OutputSignals=EQ4_LH.EQ4_LH_ELEM,EQ4_LH.EQ4_LH_HDR
  Bus Selector1 : BusSelector  OutputSignals=LSM_HWA.RoadWidth
  Bus Selector2 : BusSelector  OutputSignals=EQ4_LA.EQ4_LA_ELEM,EQ4_LA.EQ4_LA_HDR,EQ4_LRE.EQ4_LRE_ELEM
  CAL : Subsystem
  CR_RSDS_Input : Subsystem
  Chassis1 : Subsystem
  Common : Subsystem  Tag=<DSModel=3_'Fusion'>
      settings: AttributesFormatString=<DSModel='Fusion'>
  Constant : Constant  Value=0
  Control1 : Subsystem
  EQ4_Lane_Pack1 : Subsystem
  Function-Call Generator{1,3..5} (4 alike) : simulink/Ports & Subsystems/Function-Call Generator  sample_time=0.02  numberOfIterations=1  DisallowWideOutput=off
  Function-Call Generator2 : simulink/Ports & Subsystems/Function-Call Generator  sample_time=0.1  numberOfIterations=1  DisallowWideOutput=off
  Function-Call Generator6 : simulink/Ports & Subsystems/Function-Call Generator  Commented=on  sample_time=0.1  numberOfIterations=1  DisallowWideOutput=off
  IDC_L3_FD1_MSG : dsmpblib/Data Outport  Priority=-10000
      settings: SourceProductName=dSPACE Model Interface Blockset
  IFC_FD{1..3,5..6} (5 alike) : dsmpblib/Data Outport  Priority=-10000
      settings: SourceProductName=dSPACE Model Interface Blockset
  IfRFM_LANES_In : dsmpblib/Data Inport  Priority=10000
      settings: SourceProductName=dSPACE Model Interface Blockset
  LPV : Subsystem
  RFM_Road : dsmpblib/Data Inport  Priority=10000
      settings: SourceProductName=dSPACE Model Interface Blockset
  Rate Transition{1..46} (46 alike) : RateTransition  Integrity=off  Deterministic=off
  Selector1 : Selector  InputPortWidth=4  IndexOptions=Index vector (dialog)  Indices=1  OutputSizes=1
  Selector2 : Selector  InputPortWidth=4  IndexOptions=Index vector (dialog)  Indices=2  OutputSizes=1
  Selector3 : Selector  InputPortWidth=4  IndexOptions=Index vector (dialog)  Indices=3  OutputSizes=1
  Selector4 : Selector  InputPortWidth=2  IndexOptions=Index vector (dialog)  Indices=1  OutputSizes=1
  Selector5 : Selector  InputPortWidth=2  IndexOptions=Index vector (dialog)  Indices=2  OutputSizes=1
  Selector6 : Selector  InputPortWidth=4  IndexOptions=Index vector (dialog)  Indices=4  OutputSizes=1
  SensorDia : Subsystem  Commented=on
  SimBCM : Subsystem
  Software-Triggered Runnable Function1 : dsmpblib/Software-Triggered Runnable Function  Commented=on
      settings: SourceProductName=dSPACE Model Interface Blockset
  Subsystem1 : Subsystem
  Subsystem3 : Subsystem
  Subsystem4 : Subsystem
  Switch : Switch  Criteria=u2 ~= 0
  TOS : Subsystem
  TOS2 : Subsystem  Commented=on
  Terminator : Terminator  Commented=on
  UDP Receive (3)\Data Received : dsmpblib/Hardware-Triggered Runnable Function
      settings: SourceProductName=dSPACE Model Interface Blockset
  UDP Receive 2\Data Received : dsmpblib/Hardware-Triggered Runnable Function
      settings: SourceProductName=dSPACE Model Interface Blockset
  UDP_Received : Subsystem
  Unit Delay{,1..6} (7 alike) : UnitDelay  SampleTime=-1  HasFrameUpgradeWarning=on
  VCANBus : dsmpblib/Data Inport  Priority=10000
      settings: SourceProductName=dSPACE Model Interface Blockset
  aeb : Subsystem  Tag=<DSModel=2_'Osm'>
      settings: AttributesFormatString=<DSModel='Osm'>
  ifLaneBus_out_In : dsmpblib/Data Inport  Priority=10000
      settings: SourceProductName=dSPACE Model Interface Blockset
  wires:
  [RoadBus] -> Rate Transition14/1  "roadbus"
  [RoadBus] -> Rate Transition38/1
  [IfCANBus] -> Rate Transition19/1
  [LATBus] -> Unit Delay1/1
  [IfVIEBus] -> aeb/2(IfVIEBus)
  Unit Delay3/1 -> Rate Transition39/1  "aebbus"
  Control1/1(IfLONBus) -> [LONBus], Rate Transition8/1
  [AEBBus] -> Unit Delay3/1
  Rate Transition18/1 -> Bus Creator/5  "lonbus"
  [IfEHRBus] -> Rate Transition36/1
  Control1/2(IfLATBus) -> Rate Transition7/1, [LATBus]
  [IfVIEBus] -> Rate Transition37/1
  [IfLineBus] -> Rate Transition35/1
  [LONBus] -> Unit Delay2/1
  aeb/1(IfAEBSBus) -> Rate Transition43/1, [AEBBus]
  Rate Transition20/1 -> Bus Creator/6  "latbus"
  [visMsg] -> Rate Transition16/1
  ifLaneBus_out_In/1 -> Subsystem4/4(lanebus)  "lanebus"
  TOS/1(IfTOSBus) -> Rate Transition10/1, Rate Transition44/1, Rate Transition34/1
  [ifVSMBus] -> Unit Delay/1
  [IfLineBus] -> Rate Transition13/1  "lanebus"
  [ifObjectBus] -> Rate Transition12/1
  [ifVSMBus] -> aeb/3(IfVSMBus)
  UDP Receive 2\Data Received/1 -> UDP_Received/Trigger
  UDP_Received/1(visMsg) -> [visMsg]
  Rate Transition16/1 -> Chassis1/11(IfVEQ4Bus)
  Unit Delay/1 -> TOS/1(IfStateMBus)
  [IfVIEBus] -> TOS/2(IfVIEBus)
  [IfCANBus] -> TOS/3(IfVCAN)
  EQ4_Lane_Pack1/2(EQ4_LA) -> Bus Creator1/2  "EQ4_LA"
  EQ4_Lane_Pack1/3(EQ4_LH) -> Bus Creator1/3  "EQ4_LH"
  EQ4_Lane_Pack1/4(EQ4_LRE) -> Bus Creator1/4  "EQ4_LRE"
  [visMsg] -> TOS/4(VisMsg)
  Bus Creator/1 -> LPV/3(IfALLBus)
  Rate Transition22/1 -> LPV/4(IfCANBus)
  Rate Transition23/1 -> LPV/6(IfDMSBus)
  [IfCANBus] -> Rate Transition22/1
  Rate Transition29/1 -> LPV/7(IfEHRBus)
  [IfDMSBus] -> Rate Transition23/1
  Rate Transition30/1 -> LPV/8(IfVIEBus)
  [IfVIEBus] -> Rate Transition30/1
  [IfEHRBus] -> Rate Transition29/1
  Rate Transition31/1 -> EQ4_Lane_Pack1/1(In1)  "visMsg"
  Rate Transition32/1 -> LPV/9(IfEQ4Bus)
  Function-Call Generator4/1 -> LPV/Trigger
  Function-Call Generator5/1 -> Control1/Trigger
  Rate Transition19/1 -> Control1/1(IfVCANBus)
  Rate Transition33/1 -> Control1/2(IfVSMBus)
  Rate Transition34/1 -> Control1/3(IfTOSBus)
  Rate Transition35/1 -> Control1/4(IfRFMBus)
  Rate Transition36/1 -> Control1/5(IfEHRBus)
  Rate Transition37/1 -> Control1/6(IfVIEBus)
  Rate Transition38/1 -> Control1/7(IfRoadBus)
  [visMsg] -> Rate Transition31/1
  LPV/2(IfLSMBus) -> [IfLSMBus]
  LPV/1(IfVSMBus) -> Rate Transition33/1, [ifVSMBus]
  Rate Transition10/1 -> Bus Creator/1
  Rate Transition12/1 -> Bus Creator/2
  Rate Transition13/1 -> Bus Creator/3  "lanebus"
  Rate Transition14/1 -> Bus Creator/4  "roadbus"
  Unit Delay2/1 -> Rate Transition18/1  "lonbus"
  Unit Delay1/1 -> Rate Transition20/1  "latbus"
  Rate Transition39/1 -> Bus Creator/7  "aebbus"
  [IfLineBus] -> Rate Transition1/1  "lanebus"
  Rate Transition1/1 -> Chassis1/14(LaneBus)  "lanebus"
  [IfCANBus] -> Rate Transition42/1
  CAL/1(IfCALBus) -> [IfCALBus]
  [IfCALBus] -> Rate Transition5/1
  Rate Transition5/1 -> LPV/5(IfCALBus)
  [IfCALBus] -> Rate Transition41/1
  [IfVIEBus] -> Rate Transition40/1
  [IfLSMBus] -> Rate Transition17/1
  [IfEHRBus] -> Rate Transition6/1
  [IfDMSBus] -> Rate Transition4/1
  Rate Transition6/1 -> Chassis1/12(IfEHRBus)
  Rate Transition4/1 -> Chassis1/13(IfDMSBus)
  [RoadBus] -> Rate Transition45/1  "roadbus"
  [ifVSMBus] -> Rate Transition26/1
  Rate Transition7/1 -> Chassis1/9(IfLatCtrlBus)
  Rate Transition8/1 -> Chassis1/8(IfLonCtrlBus)
  Rate Transition17/1 -> Chassis1/7(IfLSMBus)
  Rate Transition26/1 -> Chassis1/6(IfVSMBus)
  Rate Transition40/1 -> Chassis1/5(IfVIEBus)
  Rate Transition41/1 -> Chassis1/4(IfCALBus)
  Rate Transition42/1 -> Chassis1/3(IfVCANBus)
  Rate Transition43/1 -> Chassis1/15(IfAEBBus)  "lanebus"
  Rate Transition44/1 -> Chassis1/16(IfOSMBus)  "lanebus"
  Rate Transition45/1 -> Chassis1/17(RoadBus)  "lanebus"
  Function-Call Generator1/1 -> Chassis1/Trigger
  Function-Call Generator3/1 -> Common/Trigger
  [IfCANBus] -> Rate Transition3/1
  Common/2(IfDMSBus) -> [IfDMSBus]
  Common/4(IfEHRBus) -> [IfEHRBus]
  Common/3(IfVIEBus) -> [IfVIEBus]
  Rate Transition3/1 -> Common/1(IfCANBus)  "lonbus"
  LPV/3(IfPlanbus) -> [ifPlanbus], Rate Transition15/1, Rate Transition9/1
  Rate Transition9/1 -> Control1/8(IfPlanbus)
  [RFM_LANES] -> Rate Transition11/1
  Rate Transition11/1 -> LPV/10(RFM_LANES)
  EQ4_Lane_Pack1/1(EQ4_LAP) -> Bus Creator1/1  "EQ4_LAP"
  Chassis1/8(ACC_FD3) -> ACC_FD4/1
  Chassis1/1(IFC_FD1) -> IFC_FD1/1
  Chassis1/2(IFC_FD2) -> IFC_FD2/1
  Chassis1/3(IFC_FD3) -> IFC_FD3/1
  Chassis1/4(IFC_FD5) -> IFC_FD5/1
  Chassis1/5(IFC_FD6) -> IFC_FD6/1
  Chassis1/6(ACC_FD1) -> ACC_FD1/1
  Chassis1/7(ACC_FD2) -> ACC_FD2/1
  Rate Transition15/1 -> Chassis1/10(IfPlanbus)
  Rate Transition21/1 -> Subsystem1/1(l3_RFMResult)  "lonbus"
  IfRFM_LANES_In/1 -> Subsystem1/3(lane)
  RFM_Road/1 -> Subsystem1/2(road)
  Subsystem1/1(IfRFM_LANES_In) -> [RFM_LANES]
  Subsystem1/2(roadbus) -> [RoadBus]  "roadbus"
  Subsystem3/1(Out2) -> Rate Transition21/1
  UDP Receive (3)\Data Received/1 -> Subsystem3/Trigger
  CR_RSDS_Input/1(LC_Obj) -> [LC_Obj]
  [LC_Obj] -> TOS/5(LC_Obj)
  Selector4/1 -> Subsystem4/1(EQ4_LH_ELEM_0)
  Selector5/1 -> Subsystem4/2(EQ4_LH_ELEM_1)
  Bus Selector/1 -> Selector5/1, Selector4/1  "<EQ4_LH_ELEM>"
  Bus Selector/2 -> Subsystem4/3(LH_HDR)  "<EQ4_LH_HDR>"
  Subsystem4/1(Out1) -> [IfLineBus]
  [IfLSMBus] -> Bus Selector1/1
  Rate Transition24/1 -> Control1/9(roadwidth)
  Bus Selector1/1 -> Rate Transition24/1  "<RoadWidth>"
  Selector6/1 -> Subsystem4/8(EQ4_LA_ELEM_3)
  Selector3/1 -> Subsystem4/7(EQ4_LA_ELEM_2)
  Bus Selector2/3 -> Subsystem4/10(In10)  "<EQ4_LRE_ELEM>"
  Bus Selector2/1 -> Selector2/1, Selector1/1, Selector3/1, Selector6/1  "<EQ4_LA_ELEM>"
  Bus Selector2/2 -> Subsystem4/9(LA_HDR)  "<EQ4_LA_HDR>"
  Selector2/1 -> Subsystem4/6(EQ4_LA_ELEM_1)
  Bus Creator1/1 -> Bus Selector2/1, Bus Selector/1, Rate Transition32/1
  Selector1/1 -> Subsystem4/5(EQ4_LA_ELEM_0)
  Chassis1/9(IDC_L3_FD1) -> IDC_L3_FD1_MSG/1
  [IfLSMBus] -> Unit Delay4/1
  Unit Delay4/1 -> Subsystem1/4(LSMback)
  SimBCM/3(CSASim_IDC_L2_LampReq) -> [CSASim_IDC_L2_LampReq]
  [ifPlanbus] -> Rate Transition2/1
  VCANBus/1 -> Switch/3, Bus Assignment/1, Rate Transition27/1
  Unit Delay5/1 -> SimBCM/2(PLAN_ALC_DECS)
  Rate Transition2/1 -> Unit Delay5/1
  Rate Transition46/1 -> Bus Assignment/3
  Rate Transition28/1 -> Bus Assignment/2
  [CSASim_IDC_L2_LampReq] -> Rate Transition25/1
  Rate Transition25/1 -> Chassis1/18(CSASim_IDC_L2_LampReq)  "lanebus"
  Function-Call Generator2/1 -> SimBCM/Trigger
  Rate Transition27/1 -> SimBCM/1(VCAN)
  SimBCM/1(LTurnLmpSwtSts) -> Rate Transition28/1
  SimBCM/2(RTurnLmpSwtSts) -> Rate Transition46/1
  Switch/1 -> [IfCANBus]
  Bus Assignment/1 -> Switch/1
  Constant/1 -> Switch/2
  SensorDia/1(Source_Dia_CRsts) -> Terminator/1
  Function-Call Generator6/1 -> SensorDia/Trigger
  Unit Delay6/1 -> TOS/6(LSM)
  [IfLSMBus] -> Unit Delay6/1
  CR_RSDS_Input/2(LC_ObjIE) -> [LC_ObjIE]
  [LC_ObjIE] -> TOS/7(LC_ObjIE)
